simulink library "pne_pne3d_generic_std"  (R2016a)
(part 2 of 7)

      mask prompts: s1 "Solver Type: settings_iMode [-]"; s2 "Solver Step Size: settings_dt [s]"; initCmd "Initialization command"; p1 "Maximum Air Spring Level [mm] export=true name=dxMax prio=1 dataSetName=susp_dummy dataClassType=susp dataClassName=$dataSetClassAirSpring$ unit='mm' description='Maximum Air Spring Level [mm]': airSpring_Axle1.dxMax [-]"; p2 "Minimum Air Spring Level [mm] export=true name=dxMin prio=1 dataSetName=susp_dummy dataClassType=susp dataClassName=$dataSetClassAirSpring$ unit='mm' description='Minimum Air Spring Level [mm]': airSpring_Axle1.dxMin [-]"; p3 "Reference Lifting Displacement for dVRef [mm] export=true name=dxRef prio=1 dataSetName=susp_dummy dataClassType=susp dataClassName=$dataSetClassAirSpring$ unit='mm' description='Reference Lifting Displacement for dVRef [mm': airSpring_Axle1.dxRef [-]"; p4 "Lifting Speed [mm/s] export=true name=vLift prio=1 dataSetName=susp_dummy dataClassType=susp dataClassName=$dataSetClassAirSpring$ unit='mm/s' description='Lifting Speed [mm/s] ': airSpring_Axle1.vLift [-]"; p5 "Lowering Speed [mm/s] export=true name=vLow prio=1 dataSetName=susp_dummy dataClassType=susp dataClassName=$dataSetClassAirSpring$ unit='mm/s' description='Lowering Speed [mm/s] ': airSpring_Axle1.vLow [-]"; p6 "Maximum Air Spring Level [mm] export=true name=dxMax prio=1 dataSetName=susp_dummy dataClassType=susp dataClassName=$dataSetClassAirSpring$ unit='mm' description='Maximum Air Spring Level [mm]': airSpring_Axle2.dxMax [-]"; p7 "Minimum Air Spring Level [mm] export=true name=dxMin prio=1 dataSetName=susp_dummy dataClassType=susp dataClassName=$dataSetClassAirSpring$ unit='mm' description='Minimum Air Spring Level [mm]': airSpring_Axle2.dxMin [-]"; p8 "Reference Lifting Displacement for dVRef [mm] export=true name=dxRef prio=1 dataSetName=susp_dummy dataClassType=susp dataClassName=$dataSetClassAirSpring$ unit='mm' description='Reference Lifting Displacement for dVRef [mm': airSpring_Axle2.dxRef [-]"; p9 "Lifting Speed [mm/s] export=true name=vLift prio=1 dataSetName=susp_dummy dataClassType=susp dataClassName=$dataSetClassAirSpring$ unit='mm/s' description='Lifting Speed [mm/s] ': airSpring_Axle2.vLift [-]"; p10 "Lowering Speed [mm/s] export=true name=vLow prio=1 dataSetName=susp_dummy dataClassType=susp dataClassName=$dataSetClassAirSpring$ unit='mm/s' description='Lowering Speed [mm/s] ': airSpring_Axle2.vLow [-]"; p11 "Maximum Air Spring Level [mm] export=true name=dxMax prio=1 dataSetName=susp_dummy dataClassType=susp dataClassName=$dataSetClassAirSpring$ unit='mm' description='Maximum Air Spring Level [mm]': airSpring_Axle3.dxMax [-]"; p12 "Minimum Air Spring Level [mm] export=true name=dxMin prio=1 dataSetName=susp_dummy dataClassType=susp dataClassName=$dataSetClassAirSpring$ unit='mm' description='Minimum Air Spring Level [mm]': airSpring_Axle3.dxMin [-]"; p13 "Reference Lifting Displacement for dVRef [mm] export=true name=dxRef prio=1 dataSetName=susp_dummy dataClassType=susp dataClassName=$dataSetClassAirSpring$ unit='mm' description='Reference Lifting Displacement for dVRef [mm': airSpring_Axle3.dxRef [-]"; p14 "Lifting Speed [mm/s] export=true name=vLift prio=1 dataSetName=susp_dummy dataClassType=susp dataClassName=$dataSetClassAirSpring$ unit='mm/s' description='Lifting Speed [mm/s] ': airSpring_Axle3.vLift [-]"; p15 "Lowering Speed [mm/s] export=true name=vLow prio=1 dataSetName=susp_dummy dataClassType=susp dataClassName=$dataSetClassAirSpring$ unit='mm/s' description='Lowering Speed [mm/s] ': airSpring_Axle3.vLow [-]"; p16 "Maximum Air Spring Level [mm] export=true name=dxMax prio=1 dataSetName=susp_dummy dataClassType=susp dataClassName=$dataSetClassAirSpring$ unit='mm' description='Maximum Air Spring Level [mm]': airSpring_Axle4.dxMax [-]"; p17 "Minimum Air Spring Level [mm] export=true name=dxMin prio=1 dataSetName=susp_dummy dataClassType=susp dataClassName=$dataSetClassAirSpring$ unit='mm' description='Minimum Air Spring Level [mm]': airSpring_Axle4.dxMin [-]"; p18 "Reference Lifting Displacement for dVRef [mm] export=true name=dxRef prio=1 dataSetName=susp_dummy dataClassType=susp dataClassName=$dataSetClassAirSpring$ unit='mm' description='Reference Lifting Displacement for dVRef [mm': airSpring_Axle4.dxRef [-]"; p19 "Lifting Speed [mm/s] export=true name=vLift prio=1 dataSetName=susp_dummy dataClassType=susp dataClassName=$dataSetClassAirSpring$ unit='mm/s' description='Lifting Speed [mm/s] ': airSpring_Axle4.vLift [-]"; p20 "Lowering Speed [mm/s] export=true name=vLow prio=1 dataSetName=susp_dummy dataClassType=susp dataClassName=$dataSetClassAirSpring$ unit='mm/s' description='Lowering Speed [mm/s] ': airSpring_Axle4.vLow [-]"; p21 "Brake Type (Disc - 0, Drum - 1)  export=true name=brakeType prio=1 dataSetName=brk_dummy dataClassType=brk dataClassName=$dataSetClassBrk$ unit='-' description='Brake Type (Disc - 0, Drum - 1)': BrakeA1_R.brakeType [-]"; p22 "brake type dependent surface area [m^2] (C_TEM_A_NORM) export=true name=bt_A_norm prio=1 dataSetName=brk_dummy dataClassType=brk dataClassName=$dataSetClassBrk$  unit='m^2' description='brake type dependent surface area [m^2] (C_TEM_A_NORM)': BrakeA1_R.bt_A_norm [m²]"; p23 "brake pad friction area [m^2] export=true name=bt_A_pad prio=1 dataSetName=brk_dummy dataClassType=brk dataClassName=$dataSetClassBrk$  unit='m^2' description='brake pad friction area [m^2]': BrakeA1_R.bt_A_pad [m²]"; p24 "brake type dependent scaling for the heat loss due to convection at the cooling brake surface [-] (C_TEM_FAC_CONV_COOL) export=true name=bt_alpha_conv_fac_cool prio=1 dataSetName=brk_dummy dataClassType=brk dataClassName=$dataSetClassBrk$  unit='-' description='bbrake type dependent scaling for the heat loss due to convection at the cooling brake surface [-] (C_TEM_FAC_CONV_COOL)': BrakeA1_R.bt_alpha_conv_fac_cool [-]"; p25 "brake type dependent scaling for the heat loss due to convection at the friction brake surface [-] (C_TEM_FAC_CONV_FRIC) export=true name=bt_alpha_conv_fac_fric prio=1 dataSetName=brk_dummy dataClassType=brk dataClassName=$dataSetClassBrk$  unit='-' description='brake type dependent scaling for the heat loss due to convection at the friction brake surface [-] (C_TEM_FAC_CONV_FRIC)': BrakeA1_R.bt_alpha_conv_fac_fric [-]"; p26 "brake type dependent correction of heat loss due to conduction into the brake base [-] (C_TEM_CONDUCT_BASE) export=true name=bt_base_conduction_corr prio=1 dataSetName=brk_dummy dataClassType=brk dataClassName=$dataSetClassBrk$  unit='-' description='brake type dependent correction of heat loss due to conduction into the brake base [-] (C_TEM_CONDUCT_BASE)': BrakeA1_R.bt_base_conduction_corr [-]"; p27 "brake type dependent spatial discretization length [m] (C_TEM_DELTA_R) export=true name=bt_delta_r prio=1 dataSetName=brk_dummy dataClassType=brk dataClassName=$dataSetClassBrk$  unit='m' description='brake type dependent spatial discretization length [m] (C_TEM_DELTA_R)': BrakeA1_R.bt_delta_r [m]"; p28 "brake type dependent density correction [-] (C_TEM_DENSITY_CORR) export=true name=bt_density_correction prio=1 dataSetName=brk_dummy dataClassType=brk dataClassName=$dataSetClassBrk$  unit='-' description='brake type dependent density correction [-] (C_TEM_DENSITY_CORR)': BrakeA1_R.bt_density_correction [-]"; p29 "brake type dependent emission number [-] (C_TEM_EPSILON_BrakeType/C_TEM_EPSILON) export=true name=bt_epsilon_corr prio=1 dataSetName=brk_dummy dataClassType=brk dataClassName=$dataSetClassBrk$  unit='-' description='brake type dependent emission number [-] (C_TEM_EPSILON_BrakeType/C_TEM_EPSILON)': BrakeA1_R.bt_epsilon_corr [-]"; p30 "brake type dependent correction for cylindrical coordinates [-] (C_TEM_CYLINDER_CORR) export=true name=bt_rad_offset prio=1 dataSetName=brk_dummy dataClassType=brk dataClassName=$dataSetClassBrk$  unit='-' description='brake type dependent correction for cylindrical coordinates [-] (C_TEM_CYLINDER_CORR)': BrakeA1_R.bt_rad_offset [-]"; p31 "brake type dependent area correction for radiation [-] (C_TEM_RAD_AREA_CORR) export=true name=bt_radiation_area_corr prio=1 dataSetName=brk_dummy dataClassType=brk dataClassName=$dataSetClassBrk$  unit='-' description='brake type dependent area correction for radiation [-] (C_TEM_RAD_AREA_CORR)': BrakeA1_R.bt_radiation_area_corr [-]"; p32 "Consider Grinding Torque (0-false, 1-true) export=true name=considerTg prio=1 dataSetName=brk_dummy dataClassType=brk dataClassName=$dataSetClassBrk$  unit='-' description='Consider Grinding Torque (0-false, 1-true)': BrakeA1_R.considerTg [-]"; p33 "Brake Factor export=true name=Cs prio=1 dataSetName=brk_dummy dataClassType=brk dataClassName=$dataSetClassBrk$  unit='-' description='Brake Factor': BrakeA1_R.Cs [-]"; p34 "Efficiency export=true name=eta prio=1 dataSetName=brk_dummy dataClassType=brk dataClassName=$dataSetClassBrk$  unit='-' description='Efficiency': BrakeA1_R.eta [-]"; p35 "Dimension Temperature Correction Factor-Vector Length (max. 25) export=true name=fac_T_Dim prio=1 dataSetName=brk_dummy dataClassType=brk dataClassName=$dataSetClassBrk$  unit='-' description='Dimension Temperature Correction Factor-Vector Length (max. 25)': BrakeA1_R.fac_T_Dim [-]"; p36 "Dimension Velocity Correction Factor-Vector Length (max. 10) export=true name=fac_v_Dim prio=1 dataSetName=brk_dummy dataClassType=brk dataClassName=$dataSetClassBrk$  unit='-' description='Dimension Velocity Correction Factor-Vector Length (max. 10)': BrakeA1_R.fac_v_Dim [-]"; p37 "Dimension Fdx-Vector Length (max. 10) export=true name=Fdx_Dim prio=1 dataSetName=brk_dummy dataClassType=brk dataClassName=$dataSetClassBrk$  unit='-' description='Dimension Fdx-Vector Length (max. 10)': BrakeA1_R.Fdx_Dim [-]"; p38 "Gathering Factor Wear export=true name=Gwear prio=1 dataSetName=brk_dummy dataClassType=brk dataClassName=$dataSetClassBrk$  unit='-' description='Gathering Factor Wear': BrakeA1_R.Gwear [-]"; p39 "Dimension of i-dx-Vector Length (Transmission Ratio FBrake/FPiston) (max. 15) export=true name=i_Dim prio=1 dataSetName=brk_dummy dataClassType=brk dataClassName=$dataSetClassBrk$  unit='-' description='Dimension of i-dx-Vector Length (Transmission Ratio FBrake/FPiston) (max. 15)': BrakeA1_R.i_Dim [-]"; p40 "Effective Brake Radius export=true name=reff prio=1 dataSetName=brk_dummy dataClassType=brk dataClassName=$dataSetClassBrk$  unit='m' description='Effective Brake Radius': BrakeA1_R.reff [m]"; p41 "Initial Sum Brake Pad Thickness sPad_sum0 export=true name=sPad_sum0 prio=1 dataSetName=brk_dummy dataClassType=brk dataClassName=$dataSetClassBrk$  unit='m' description='Initial Sum Brake Pad Thickness sPad_sum0 [m]': BrakeA1_R.sPad_sum0 [m]"; p42 "Temperature calculation mode: 0 - constant temperature, 1 - variable temperature export=true name=useVarTempCalc prio=1 dataSetName=brk_dummy dataClassType=brk dataClassName=$dataSetClassBrk$  unit='-' description='Temperature calculation mode: 0 - constant temperature, 1 - variable temperature': BrakeA1_R.useVarTempCalc [-]"; p43 "Dimension Temperature Correction Factor-Vector Length (max. 20) export=true name=wearRate_T_Dim prio=1 dataSetName=brk_dummy dataClassType=brk dataClassName=$dataSetClassBrk$  unit='-' description='Dimension Temperature Correction Factor-Vector Length (max. 20)': BrakeA1_R.wearRate_T_Dim [-]"; p44 "Brake Type (Disc - 0, Drum - 1)  export=true name=brakeType prio=1 dataSetName=brk_dummy dataClassType=brk dataClassName=$dataSetClassBrk$ unit='-' description='Brake Type (Disc - 0, Drum - 1)': BrakeA2_R.brakeType [-]"; p45 "brake type dependent surface area [m^2] (C_TEM_A_NORM) export=true name=bt_A_norm prio=1 dataSetName=brk_dummy dataClassType=brk dataClassName=$dataSetClassBrk$  unit='m^2' description='brake type dependent surface area [m^2] (C_TEM_A_NORM)': BrakeA2_R.bt_A_norm [m²]"; p46 "brake pad friction area [m^2] export=true name=bt_A_pad prio=1 dataSetName=brk_dummy dataClassType=brk dataClassName=$dataSetClassBrk$  unit='m^2' description='brake pad friction area [m^2]': BrakeA2_R.bt_A_pad [m²]"; p47 "brake type dependent scaling for the heat loss due to convection at the cooling brake surface [-] (C_TEM_FAC_CONV_COOL) export=true name=bt_alpha_conv_fac_cool prio=1 dataSetName=brk_dummy dataClassType=brk dataClassName=$dataSetClassBrk$  unit='-' description='bbrake type dependent scaling for the heat loss due to convection at the cooling brake surface [-] (C_TEM_FAC_CONV_COOL)': BrakeA2_R.bt_alpha_conv_fac_cool [-]"; p48 "brake type dependent scaling for the heat loss due to convection at the friction brake surface [-] (C_TEM_FAC_CONV_FRIC) export=true name=bt_alpha_conv_fac_fric prio=1 dataSetName=brk_dummy dataClassType=brk dataClassName=$dataSetClassBrk$  unit='-' description='brake type dependent scaling for the heat loss due to convection at the friction brake surface [-] (C_TEM_FAC_CONV_FRIC)': BrakeA2_R.bt_alpha_conv_fac_fric [-]"; p49 "brake type dependent correction of heat loss due to conduction into the brake base [-] (C_TEM_CONDUCT_BASE) export=true name=bt_base_conduction_corr prio=1 dataSetName=brk_dummy dataClassType=brk dataClassName=$dataSetClassBrk$  unit='-' description='brake type dependent correction of heat loss due to conduction into the brake base [-] (C_TEM_CONDUCT_BASE)': BrakeA2_R.bt_base_conduction_corr [-]"; p50 "brake type dependent spatial discretization length [m] (C_TEM_DELTA_R) export=true name=bt_delta_r prio=1 dataSetName=brk_dummy dataClassType=brk dataClassName=$dataSetClassBrk$  unit='m' description='brake type dependent spatial discretization length [m] (C_TEM_DELTA_R)': BrakeA2_R.bt_delta_r [m]"; p51 "brake type dependent density correction [-] (C_TEM_DENSITY_CORR) export=true name=bt_density_correction prio=1 dataSetName=brk_dummy dataClassType=brk dataClassName=$dataSetClassBrk$  unit='-' description='brake type dependent density correction [-] (C_TEM_DENSITY_CORR)': BrakeA2_R.bt_density_correction [-]"; p52 "brake type dependent emission number [-] (C_TEM_EPSILON_BrakeType/C_TEM_EPSILON) export=true name=bt_epsilon_corr prio=1 dataSetName=brk_dummy dataClassType=brk dataClassName=$dataSetClassBrk$  unit='-' description='brake type dependent emission number [-] (C_TEM_EPSILON_BrakeType/C_TEM_EPSILON)': BrakeA2_R.bt_epsilon_corr [-]"; p53 "brake type dependent correction for cylindrical coordinates [-] (C_TEM_CYLINDER_CORR) export=true name=bt_rad_offset prio=1 dataSetName=brk_dummy dataClassType=brk dataClassName=$dataSetClassBrk$  unit='-' description='brake type dependent correction for cylindrical coordinates [-] (C_TEM_CYLINDER_CORR)': BrakeA2_R.bt_rad_offset [-]"; p54 "brake type dependent area correction for radiation [-] (C_TEM_RAD_AREA_CORR) export=true name=bt_radiation_area_corr prio=1 dataSetName=brk_dummy dataClassType=brk dataClassName=$dataSetClassBrk$  unit='-' description='brake type dependent area correction for radiation [-] (C_TEM_RAD_AREA_CORR)': BrakeA2_R.bt_radiation_area_corr [-]"; p55 "Consider Grinding Torque (0-false, 1-true) export=true name=considerTg prio=1 dataSetName=brk_dummy dataClassType=brk dataClassName=$dataSetClassBrk$  unit='-' description='Consider Grinding Torque (0-false, 1-true)': BrakeA2_R.considerTg [-]"; p56 "Brake Factor export=true name=Cs prio=1 dataSetName=brk_dummy dataClassType=brk dataClassName=$dataSetClassBrk$  unit='-' description='Brake Factor': BrakeA2_R.Cs [-]"; p57 "Efficiency export=true name=eta prio=1 dataSetName=brk_dummy dataClassType=brk dataClassName=$dataSetClassBrk$  unit='-' description='Efficiency': BrakeA2_R.eta [-]"; p58 "Dimension Temperature Correction Factor-Vector Length (max. 25) export=true name=fac_T_Dim prio=1 dataSetName=brk_dummy dataClassType=brk dataClassName=$dataSetClassBrk$  unit='-' description='Dimension Temperature Correction Factor-Vector Length (max. 25)': BrakeA2_R.fac_T_Dim [-]"; p59 "Dimension Velocity Correction Factor-Vector Length (max. 10) export=true name=fac_v_Dim prio=1 dataSetName=brk_dummy dataClassType=brk dataClassName=$dataSetClassBrk$  unit='-' description='Dimension Velocity Correction Factor-Vector Length (max. 10)': BrakeA2_R.fac_v_Dim [-]"; p60 "Dimension Fdx-Vector Length (max. 10) export=true name=Fdx_Dim prio=1 dataSetName=brk_dummy dataClassType=brk dataClassName=$dataSetClassBrk$  unit='-' description='Dimension Fdx-Vector Length (max. 10)': BrakeA2_R.Fdx_Dim [-]"; p61 "Gathering Factor Wear export=true name=Gwear prio=1 dataSetName=brk_dummy dataClassType=brk dataClassName=$dataSetClassBrk$  unit='-' description='Gathering Factor Wear': BrakeA2_R.Gwear [-]"; p62 "Dimension of i-dx-Vector Length (Transmission Ratio FBrake/FPiston) (max. 15) export=true name=i_Dim prio=1 dataSetName=brk_dummy dataClassType=brk dataClassName=$dataSetClassBrk$  unit='-' description='Dimension of i-dx-Vector Length (Transmission Ratio FBrake/FPiston) (max. 15)': BrakeA2_R.i_Dim [-]"; p63 "Effective Brake Radius export=true name=reff prio=1 dataSetName=brk_dummy dataClassType=brk dataClassName=$dataSetClassBrk$  unit='m' description='Effective Brake Radius': BrakeA2_R.reff [m]"; p64 "Initial Sum Brake Pad Thickness sPad_sum0 export=true name=sPad_sum0 prio=1 dataSetName=brk_dummy dataClassType=brk dataClassName=$dataSetClassBrk$  unit='m' description='Initial Sum Brake Pad Thickness sPad_sum0 [m]': BrakeA2_R.sPad_sum0 [m]"; p65 "Temperature calculation mode: 0 - constant temperature, 1 - variable temperature export=true name=useVarTempCalc prio=1 dataSetName=brk_dummy dataClassType=brk dataClassName=$dataSetClassBrk$  unit='-' description='Temperature calculation mode: 0 - constant temperature, 1 - variable temperature': BrakeA2_R.useVarTempCalc [-]"; p66 "Dimension Temperature Correction Factor-Vector Length (max. 20) export=true name=wearRate_T_Dim prio=1 dataSetName=brk_dummy dataClassType=brk dataClassName=$dataSetClassBrk$  unit='-' description='Dimension Temperature Correction Factor-Vector Length (max. 20)': BrakeA2_R.wearRate_T_Dim [-]"; p67 "Brake Type (Disc - 0, Drum - 1)  export=true name=brakeType prio=1 dataSetName=brk_dummy dataClassType=brk dataClassName=$dataSetClassBrk$ unit='-' description='Brake Type (Disc - 0, Drum - 1)': BrakeA3_R.brakeType [-]"; p68 "brake type dependent surface area [m^2] (C_TEM_A_NORM) export=true name=bt_A_norm prio=1 dataSetName=brk_dummy dataClassType=brk dataClassName=$dataSetClassBrk$  unit='m^2' description='brake type dependent surface area [m^2] (C_TEM_A_NORM)': BrakeA3_R.bt_A_norm [m²]"; p69 "brake pad friction area [m^2] export=true name=bt_A_pad prio=1 dataSetName=brk_dummy dataClassType=brk dataClassName=$dataSetClassBrk$  unit='m^2' description='brake pad friction area [m^2]': BrakeA3_R.bt_A_pad [m²]"; p70 "brake type dependent scaling for the heat loss due to convection at the cooling brake surface [-] (C_TEM_FAC_CONV_COOL) export=true name=bt_alpha_conv_fac_cool prio=1 dataSetName=brk_dummy dataClassType=brk dataClassName=$dataSetClassBrk$  unit='-' description='bbrake type dependent scaling for the heat loss due to convection at the cooling brake surface [-] (C_TEM_FAC_CONV_COOL)': BrakeA3_R.bt_alpha_conv_fac_cool [-]"; p71 "brake type dependent scaling for the heat loss due to convection at the friction brake surface [-] (C_TEM_FAC_CONV_FRIC) export=true name=bt_alpha_conv_fac_fric prio=1 dataSetName=brk_dummy dataClassType=brk dataClassName=$dataSetClassBrk$  unit='-' description='brake type dependent scaling for the heat loss due to convection at the friction brake surface [-] (C_TEM_FAC_CONV_FRIC)': BrakeA3_R.bt_alpha_conv_fac_fric [-]"; p72 "brake type dependent correction of heat loss due to conduction into the brake base [-] (C_TEM_CONDUCT_BASE) export=true name=bt_base_conduction_corr prio=1 dataSetName=brk_dummy dataClassType=brk dataClassName=$dataSetClassBrk$  unit='-' description='brake type dependent correction of heat loss due to conduction into the brake base [-] (C_TEM_CONDUCT_BASE)': BrakeA3_R.bt_base_conduction_corr [-]"; p73 "brake type dependent spatial discretization length [m] (C_TEM_DELTA_R) export=true name=bt_delta_r prio=1 dataSetName=brk_dummy dataClassType=brk dataClassName=$dataSetClassBrk$  unit='m' description='brake type dependent spatial discretization length [m] (C_TEM_DELTA_R)': BrakeA3_R.bt_delta_r [m]"; p74 "brake type dependent density correction [-] (C_TEM_DENSITY_CORR) export=true name=bt_density_correction prio=1 dataSetName=brk_dummy dataClassType=brk dataClassName=$dataSetClassBrk$  unit='-' description='brake type dependent density correction [-] (C_TEM_DENSITY_CORR)': BrakeA3_R.bt_density_correction [-]"; p75 "brake type dependent emission number [-] (C_TEM_EPSILON_BrakeType/C_TEM_EPSILON) export=true name=bt_epsilon_corr prio=1 dataSetName=brk_dummy dataClassType=brk dataClassName=$dataSetClassBrk$  unit='-' description='brake type dependent emission number [-] (C_TEM_EPSILON_BrakeType/C_TEM_EPSILON)': BrakeA3_R.bt_epsilon_corr [-]"; p76 "brake type dependent correction for cylindrical coordinates [-] (C_TEM_CYLINDER_CORR) export=true name=bt_rad_offset prio=1 dataSetName=brk_dummy dataClassType=brk dataClassName=$dataSetClassBrk$  unit='-' description='brake type dependent correction for cylindrical coordinates [-] (C_TEM_CYLINDER_CORR)': BrakeA3_R.bt_rad_offset [-]"; p77 "brake type dependent area correction for radiation [-] (C_TEM_RAD_AREA_CORR) export=true name=bt_radiation_area_corr prio=1 dataSetName=brk_dummy dataClassType=brk dataClassName=$dataSetClassBrk$  unit='-' description='brake type dependent area correction for radiation [-] (C_TEM_RAD_AREA_CORR)': BrakeA3_R.bt_radiation_area_corr [-]"; p78 "Consider Grinding Torque (0-false, 1-true) export=true name=considerTg prio=1 dataSetName=brk_dummy dataClassType=brk dataClassName=$dataSetClassBrk$  unit='-' description='Consider Grinding Torque (0-false, 1-true)': BrakeA3_R.considerTg [-]"; p79 "Brake Factor export=true name=Cs prio=1 dataSetName=brk_dummy dataClassType=brk dataClassName=$dataSetClassBrk$  unit='-' description='Brake Factor': BrakeA3_R.Cs [-]"; p80 "Efficiency export=true name=eta prio=1 dataSetName=brk_dummy dataClassType=brk dataClassName=$dataSetClassBrk$  unit='-' description='Efficiency': BrakeA3_R.eta [-]"; p81 "Dimension Temperature Correction Factor-Vector Length (max. 25) export=true name=fac_T_Dim prio=1 dataSetName=brk_dummy dataClassType=brk dataClassName=$dataSetClassBrk$  unit='-' description='Dimension Temperature Correction Factor-Vector Length (max. 25)': BrakeA3_R.fac_T_Dim [-]"; p82 "Dimension Velocity Correction Factor-Vector Length (max. 10) export=true name=fac_v_Dim prio=1 dataSetName=brk_dummy dataClassType=brk dataClassName=$dataSetClassBrk$  unit='-' description='Dimension Velocity Correction Factor-Vector Length (max. 10)': BrakeA3_R.fac_v_Dim [-]"; p83 "Dimension Fdx-Vector Length (max. 10) export=true name=Fdx_Dim prio=1 dataSetName=brk_dummy dataClassType=brk dataClassName=$dataSetClassBrk$  unit='-' description='Dimension Fdx-Vector Length (max. 10)': BrakeA3_R.Fdx_Dim [-]"; p84 "Gathering Factor Wear export=true name=Gwear prio=1 dataSetName=brk_dummy dataClassType=brk dataClassName=$dataSetClassBrk$  unit='-' description='Gathering Factor Wear': BrakeA3_R.Gwear [-]"; p85 "Dimension of i-dx-Vector Length (Transmission Ratio FBrake/FPiston) (max. 15) export=true name=i_Dim prio=1 dataSetName=brk_dummy dataClassType=brk dataClassName=$dataSetClassBrk$  unit='-' description='Dimension of i-dx-Vector Length (Transmission Ratio FBrake/FPiston) (max. 15)': BrakeA3_R.i_Dim [-]"; p86 "Effective Brake Radius export=true name=reff prio=1 dataSetName=brk_dummy dataClassType=brk dataClassName=$dataSetClassBrk$  unit='m' description='Effective Brake Radius': BrakeA3_R.reff [m]"; p87 "Initial Sum Brake Pad Thickness sPad_sum0 export=true name=sPad_sum0 prio=1 dataSetName=brk_dummy dataClassType=brk dataClassName=$dataSetClassBrk$  unit='m' description='Initial Sum Brake Pad Thickness sPad_sum0 [m]': BrakeA3_R.sPad_sum0 [m]"; p88 "Temperature calculation mode: 0 - constant temperature, 1 - variable temperature export=true name=useVarTempCalc prio=1 dataSetName=brk_dummy dataClassType=brk dataClassName=$dataSetClassBrk$  unit='-' description='Temperature calculation mode: 0 - constant temperature, 1 - variable temperature': BrakeA3_R.useVarTempCalc [-]"; p89 "Dimension Temperature Correction Factor-Vector Length (max. 20) export=true name=wearRate_T_Dim prio=1 dataSetName=brk_dummy dataClassType=brk dataClassName=$dataSetClassBrk$  unit='-' description='Dimension Temperature Correction Factor-Vector Length (max. 20)': BrakeA3_R.wearRate_T_Dim [-]"; p90 "Brake Type (Disc - 0, Drum - 1)  export=true name=brakeType prio=1 dataSetName=brk_dummy dataClassType=brk dataClassName=$dataSetClassBrk$ unit='-' description='Brake Type (Disc - 0, Drum - 1)': BrakeA4_R.brakeType [-]"; p91 "brake type dependent surface area [m^2] (C_TEM_A_NORM) export=true name=bt_A_norm prio=1 dataSetName=brk_dummy dataClassType=brk dataClassName=$dataSetClassBrk$  unit='m^2' description='brake type dependent surface area [m^2] (C_TEM_A_NORM)': BrakeA4_R.bt_A_norm [m²]"; p92 "brake pad friction area [m^2] export=true name=bt_A_pad prio=1 dataSetName=brk_dummy dataClassType=brk dataClassName=$dataSetClassBrk$  unit='m^2' description='brake pad friction area [m^2]': BrakeA4_R.bt_A_pad [m²]"; p93 "brake type dependent scaling for the heat loss due to convection at the cooling brake surface [-] (C_TEM_FAC_CONV_COOL) export=true name=bt_alpha_conv_fac_cool prio=1 dataSetName=brk_dummy dataClassType=brk dataClassName=$dataSetClassBrk$  unit='-' description='bbrake type dependent scaling for the heat loss due to convection at the cooling brake surface [-] (C_TEM_FAC_CONV_COOL)': BrakeA4_R.bt_alpha_conv_fac_cool [-]"; p94 "brake type dependent scaling for the heat loss due to convection at the friction brake surface [-] (C_TEM_FAC_CONV_FRIC) export=true name=bt_alpha_conv_fac_fric prio=1 dataSetName=brk_dummy dataClassType=brk dataClassName=$dataSetClassBrk$  unit='-' description='brake type dependent scaling for the heat loss due to convection at the friction brake surface [-] (C_TEM_FAC_CONV_FRIC)': BrakeA4_R.bt_alpha_conv_fac_fric [-]"; p95 "brake type dependent correction of heat loss due to conduction into the brake base [-] (C_TEM_CONDUCT_BASE) export=true name=bt_base_conduction_corr prio=1 dataSetName=brk_dummy dataClassType=brk dataClassName=$dataSetClassBrk$  unit='-' description='brake type dependent correction of heat loss due to conduction into the brake base [-] (C_TEM_CONDUCT_BASE)': BrakeA4_R.bt_base_conduction_corr [-]"; p96 "brake type dependent spatial discretization length [m] (C_TEM_DELTA_R) export=true name=bt_delta_r prio=1 dataSetName=brk_dummy dataClassType=brk dataClassName=$dataSetClassBrk$  unit='m' description='brake type dependent spatial discretization length [m] (C_TEM_DELTA_R)': BrakeA4_R.bt_delta_r [m]"; p97 "brake type dependent density correction [-] (C_TEM_DENSITY_CORR) export=true name=bt_density_correction prio=1 dataSetName=brk_dummy dataClassType=brk dataClassName=$dataSetClassBrk$  unit='-' description='brake type dependent density correction [-] (C_TEM_DENSITY_CORR)': BrakeA4_R.bt_density_correction [-]"; p98 "brake type dependent emission number [-] (C_TEM_EPSILON_BrakeType/C_TEM_EPSILON) export=true name=bt_epsilon_corr prio=1 dataSetName=brk_dummy dataClassType=brk dataClassName=$dataSetClassBrk$  unit='-' description='brake type dependent emission number [-] (C_TEM_EPSILON_BrakeType/C_TEM_EPSILON)': BrakeA4_R.bt_epsilon_corr [-]"; p99 "brake type dependent correction for cylindrical coordinates [-] (C_TEM_CYLINDER_CORR) export=true name=bt_rad_offset prio=1 dataSetName=brk_dummy dataClassType=brk dataClassName=$dataSetClassBrk$  unit='-' description='brake type dependent correction for cylindrical coordinates [-] (C_TEM_CYLINDER_CORR)': BrakeA4_R.bt_rad_offset [-]"; p100 "brake type dependent area correction for radiation [-] (C_TEM_RAD_AREA_CORR) export=true name=bt_radiation_area_corr prio=1 dataSetName=brk_dummy dataClassType=brk dataClassName=$dataSetClassBrk$  unit='-' description='brake type dependent area correction for radiation [-] (C_TEM_RAD_AREA_CORR)': BrakeA4_R.bt_radiation_area_corr [-]"; p101 "Consider Grinding Torque (0-false, 1-true) export=true name=considerTg prio=1 dataSetName=brk_dummy dataClassType=brk dataClassName=$dataSetClassBrk$  unit='-' description='Consider Grinding Torque (0-false, 1-true)': BrakeA4_R.considerTg [-]"; p102 "Brake Factor export=true name=Cs prio=1 dataSetName=brk_dummy dataClassType=brk dataClassName=$dataSetClassBrk$  unit='-' description='Brake Factor': BrakeA4_R.Cs [-]"; p103 "Efficiency export=true name=eta prio=1 dataSetName=brk_dummy dataClassType=brk dataClassName=$dataSetClassBrk$  unit='-' description='Efficiency': BrakeA4_R.eta [-]"; p104 "Dimension Temperature Correction Factor-Vector Length (max. 25) export=true name=fac_T_Dim prio=1 dataSetName=brk_dummy dataClassType=brk dataClassName=$dataSetClassBrk$  unit='-' description='Dimension Temperature Correction Factor-Vector Length (max. 25)': BrakeA4_R.fac_T_Dim [-]"; p105 "Dimension Velocity Correction Factor-Vector Length (max. 10) export=true name=fac_v_Dim prio=1 dataSetName=brk_dummy dataClassType=brk dataClassName=$dataSetClassBrk$  unit='-' description='Dimension Velocity Correction Factor-Vector Length (max. 10)': BrakeA4_R.fac_v_Dim [-]"; p106 "Dimension Fdx-Vector Length (max. 10) export=true name=Fdx_Dim prio=1 dataSetName=brk_dummy dataClassType=brk dataClassName=$dataSetClassBrk$  unit='-' description='Dimension Fdx-Vector Length (max. 10)': BrakeA4_R.Fdx_Dim [-]"; p107 "Gathering Factor Wear export=true name=Gwear prio=1 dataSetName=brk_dummy dataClassType=brk dataClassName=$dataSetClassBrk$  unit='-' description='Gathering Factor Wear': BrakeA4_R.Gwear [-]"; p108 "Dimension of i-dx-Vector Length (Transmission Ratio FBrake/FPiston) (max. 15) export=true name=i_Dim prio=1 dataSetName=brk_dummy dataClassType=brk dataClassName=$dataSetClassBrk$  unit='-' description='Dimension of i-dx-Vector Length (Transmission Ratio FBrake/FPiston) (max. 15)': BrakeA4_R.i_Dim [-]"; p109 "Effective Brake Radius export=true name=reff prio=1 dataSetName=brk_dummy dataClassType=brk dataClassName=$dataSetClassBrk$  unit='m' description='Effective Brake Radius': BrakeA4_R.reff [m]"; p110 "Initial Sum Brake Pad Thickness sPad_sum0 export=true name=sPad_sum0 prio=1 dataSetName=brk_dummy dataClassType=brk dataClassName=$dataSetClassBrk$  unit='m' description='Initial Sum Brake Pad Thickness sPad_sum0 [m]': BrakeA4_R.sPad_sum0 [m]"; p111 "Temperature calculation mode: 0 - constant temperature, 1 - variable temperature export=true name=useVarTempCalc prio=1 dataSetName=brk_dummy dataClassType=brk dataClassName=$dataSetClassBrk$  unit='-' description='Temperature calculation mode: 0 - constant temperature, 1 - variable temperature': BrakeA4_R.useVarTempCalc [-]"; p112 "Dimension Temperature Correction Factor-Vector Length (max. 20) export=true name=wearRate_T_Dim prio=1 dataSetName=brk_dummy dataClassType=brk dataClassName=$dataSetClassBrk$  unit='-' description='Dimension Temperature Correction Factor-Vector Length (max. 20)': BrakeA4_R.wearRate_T_Dim [-]"; p113 "Dimension of Parking Brake Spring Curve (max 10) export=true name=dxFSpring_Dim prio=1 dataSetName=cyl_dummy dataClassType=cyl dataClassName=$dataSetClassCyl$  unit='-' description='Dimension of Parking Brake Spring Curve (max 10)': brakeCylinderA1_R.dxFSpring_Dim [-]"; p114 "Dimension of Parking Brake Chamber Volume Curve (max 10) export=true name=dxVolPB_Dim prio=1 dataSetName=cyl_dummy dataClassType=cyl dataClassName=$dataSetClassCyl$  unit='-' description='Dimension of Parking Brake Chamber Volume Curve (max 10)': brakeCylinderA1_R.dxVolPB_Dim [-]"; p115 "Dimension of Service Brake Chamber Volume Curve (max 10) export=true name=dxVolSB_Dim prio=1 dataSetName=cyl_dummy dataClassType=cyl dataClassName=$dataSetClassCyl$  unit='-' description='Dimension of Service Brake Chamber Volume Curve (max 10)': brakeCylinderA1_R.dxVolSB_Dim [-]"; p116 "Nominal Force Membrane Cylinder at pNom export=true name=FNom prio=1 dataSetName=cyl_dummy dataClassType=cyl dataClassName=$dataSetClassCyl$ unit='N' description='Nominal Force Membrane Cylinder at pNom': brakeCylinderA1_R.FNom [N]"; p117 "Maximum Cylinder Stroke export=true name=maxStroke prio=1 dataSetName=cyl_dummy dataClassType=cyl dataClassName=$dataSetClassCyl$ unit='m' description='Maximum Cylinder Stroke': brakeCylinderA1_R.maxStroke [m]"; p118 "Application Pressure Membrane Chamber (relative to pAtm) export=true name=pApp prio=1 dataSetName=cyl_dummy dataClassType=cyl dataClassName=$dataSetClassCyl$  unit='Pa' description='Application Pressure Membrane Chamber (relative to pAtm)': brakeCylinderA1_R.pApp [Pa]"; p119 "Nominal Pressure (relative to pAtm) export=true name=pNom prio=1 dataSetName=cyl_dummy dataClassType=cyl dataClassName=$dataSetClassCyl$ unit='Pa' description='Nominal Pressure (relative to pAtm)': brakeCylinderA1_R.pNom [Pa]"; p120 "Spring Brake Release Pressure (relative to pAtm) export=true name=pR_PB prio=1 dataSetName=cyl_dummy dataClassType=cyl dataClassName=$dataSetClassCyl$ unit='Pa' description='Spring Brake Release Pressure (relative to pAtm)': brakeCylinderA1_R.pR_PB [Pa]"; p121 "Spring Brake Release Stroke at pR_PB export=true name=xR_PB prio=1 dataSetName=cyl_dummy dataClassType=cyl dataClassName=$dataSetClassCyl$ unit='m' description='Spring Brake Release Stroke at pR_PB': brakeCylinderA1_R.xR_PB [m]"; p122 "Dimension of Parking Brake Spring Curve (max 10) export=true name=dxFSpring_Dim prio=1 dataSetName=cyl_dummy dataClassType=cyl dataClassName=$dataSetClassCyl$  unit='-' description='Dimension of Parking Brake Spring Curve (max 10)': brakeCylinderA2_R.dxFSpring_Dim [-]"; p123 "Dimension of Parking Brake Chamber Volume Curve (max 10) export=true name=dxVolPB_Dim prio=1 dataSetName=cyl_dummy dataClassType=cyl dataClassName=$dataSetClassCyl$  unit='-' description='Dimension of Parking Brake Chamber Volume Curve (max 10)': brakeCylinderA2_R.dxVolPB_Dim [-]"; p124 "Dimension of Service Brake Chamber Volume Curve (max 10) export=true name=dxVolSB_Dim prio=1 dataSetName=cyl_dummy dataClassType=cyl dataClassName=$dataSetClassCyl$  unit='-' description='Dimension of Service Brake Chamber Volume Curve (max 10)': brakeCylinderA2_R.dxVolSB_Dim [-]"; p125 "Nominal Force Membrane Cylinder at pNom export=true name=FNom prio=1 dataSetName=cyl_dummy dataClassType=cyl dataClassName=$dataSetClassCyl$ unit='N' description='Nominal Force Membrane Cylinder at pNom': brakeCylinderA2_R.FNom [N]"; p126 "Maximum Cylinder Stroke export=true name=maxStroke prio=1 dataSetName=cyl_dummy dataClassType=cyl dataClassName=$dataSetClassCyl$ unit='m' description='Maximum Cylinder Stroke': brakeCylinderA2_R.maxStroke [m]"; p127 "Application Pressure Membrane Chamber (relative to pAtm) export=true name=pApp prio=1 dataSetName=cyl_dummy dataClassType=cyl dataClassName=$dataSetClassCyl$  unit='Pa' description='Application Pressure Membrane Chamber (relative to pAtm)': brakeCylinderA2_R.pApp [Pa]"; p128 "Nominal Pressure (relative to pAtm) export=true name=pNom prio=1 dataSetName=cyl_dummy dataClassType=cyl dataClassName=$dataSetClassCyl$ unit='Pa' description='Nominal Pressure (relative to pAtm)': brakeCylinderA2_R.pNom [Pa]"; p129 "Spring Brake Release Pressure (relative to pAtm) export=true name=pR_PB prio=1 dataSetName=cyl_dummy dataClassType=cyl dataClassName=$dataSetClassCyl$ unit='Pa' description='Spring Brake Release Pressure (relative to pAtm)': brakeCylinderA2_R.pR_PB [Pa]"; p130 "Spring Brake Release Stroke at pR_PB export=true name=xR_PB prio=1 dataSetName=cyl_dummy dataClassType=cyl dataClassName=$dataSetClassCyl$ unit='m' description='Spring Brake Release Stroke at pR_PB': brakeCylinderA2_R.xR_PB [m]"; p131 "Dimension of Parking Brake Spring Curve (max 10) export=true name=dxFSpring_Dim prio=1 dataSetName=cyl_dummy dataClassType=cyl dataClassName=$dataSetClassCyl$  unit='-' description='Dimension of Parking Brake Spring Curve (max 10)': brakeCylinderA3_R.dxFSpring_Dim [-]"; p132 "Dimension of Parking Brake Chamber Volume Curve (max 10) export=true name=dxVolPB_Dim prio=1 dataSetName=cyl_dummy dataClassType=cyl dataClassName=$dataSetClassCyl$  unit='-' description='Dimension of Parking Brake Chamber Volume Curve (max 10)': brakeCylinderA3_R.dxVolPB_Dim [-]"; p133 "Dimension of Service Brake Chamber Volume Curve (max 10) export=true name=dxVolSB_Dim prio=1 dataSetName=cyl_dummy dataClassType=cyl dataClassName=$dataSetClassCyl$  unit='-' description='Dimension of Service Brake Chamber Volume Curve (max 10)': brakeCylinderA3_R.dxVolSB_Dim [-]"; p134 "Nominal Force Membrane Cylinder at pNom export=true name=FNom prio=1 dataSetName=cyl_dummy dataClassType=cyl dataClassName=$dataSetClassCyl$ unit='N' description='Nominal Force Membrane Cylinder at pNom': brakeCylinderA3_R.FNom [N]"; p135 "Maximum Cylinder Stroke export=true name=maxStroke prio=1 dataSetName=cyl_dummy dataClassType=cyl dataClassName=$dataSetClassCyl$ unit='m' description='Maximum Cylinder Stroke': brakeCylinderA3_R.maxStroke [m]"; p136 "Application Pressure Membrane Chamber (relative to pAtm) export=true name=pApp prio=1 dataSetName=cyl_dummy dataClassType=cyl dataClassName=$dataSetClassCyl$  unit='Pa' description='Application Pressure Membrane Chamber (relative to pAtm)': brakeCylinderA3_R.pApp [Pa]"; p137 "Nominal Pressure (relative to pAtm) export=true name=pNom prio=1 dataSetName=cyl_dummy dataClassType=cyl dataClassName=$dataSetClassCyl$ unit='Pa' description='Nominal Pressure (relative to pAtm)': brakeCylinderA3_R.pNom [Pa]"; p138 "Spring Brake Release Pressure (relative to pAtm) export=true name=pR_PB prio=1 dataSetName=cyl_dummy dataClassType=cyl dataClassName=$dataSetClassCyl$ unit='Pa' description='Spring Brake Release Pressure (relative to pAtm)': brakeCylinderA3_R.pR_PB [Pa]"; p139 "Spring Brake Release Stroke at pR_PB export=true name=xR_PB prio=1 dataSetName=cyl_dummy dataClassType=cyl dataClassName=$dataSetClassCyl$ unit='m' description='Spring Brake Release Stroke at pR_PB': brakeCylinderA3_R.xR_PB [m]"; p140 "Dimension of Parking Brake Spring Curve (max 10) export=true name=dxFSpring_Dim prio=1 dataSetName=cyl_dummy dataClassType=cyl dataClassName=$dataSetClassCyl$  unit='-' description='Dimension of Parking Brake Spring Curve (max 10)': brakeCylinderA4_R.dxFSpring_Dim [-]"; p141 "Dimension of Parking Brake Chamber Volume Curve (max 10) export=true name=dxVolPB_Dim prio=1 dataSetName=cyl_dummy dataClassType=cyl dataClassName=$dataSetClassCyl$  unit='-' description='Dimension of Parking Brake Chamber Volume Curve (max 10)': brakeCylinderA4_R.dxVolPB_Dim [-]"; p142 "Dimension of Service Brake Chamber Volume Curve (max 10) export=true name=dxVolSB_Dim prio=1 dataSetName=cyl_dummy dataClassType=cyl dataClassName=$dataSetClassCyl$  unit='-' description='Dimension of Service Brake Chamber Volume Curve (max 10)': brakeCylinderA4_R.dxVolSB_Dim [-]"; p143 "Nominal Force Membrane Cylinder at pNom export=true name=FNom prio=1 dataSetName=cyl_dummy dataClassType=cyl dataClassName=$dataSetClassCyl$ unit='N' description='Nominal Force Membrane Cylinder at pNom': brakeCylinderA4_R.FNom [N]"; p144 "Maximum Cylinder Stroke export=true name=maxStroke prio=1 dataSetName=cyl_dummy dataClassType=cyl dataClassName=$dataSetClassCyl$ unit='m' description='Maximum Cylinder Stroke': brakeCylinderA4_R.maxStroke [m]"; p145 "Application Pressure Membrane Chamber (relative to pAtm) export=true name=pApp prio=1 dataSetName=cyl_dummy dataClassType=cyl dataClassName=$dataSetClassCyl$  unit='Pa' description='Application Pressure Membrane Chamber (relative to pAtm)': brakeCylinderA4_R.pApp [Pa]"; p146 "Nominal Pressure (relative to pAtm) export=true name=pNom prio=1 dataSetName=cyl_dummy dataClassType=cyl dataClassName=$dataSetClassCyl$ unit='Pa' description='Nominal Pressure (relative to pAtm)': brakeCylinderA4_R.pNom [Pa]"; p147 "Spring Brake Release Pressure (relative to pAtm) export=true name=pR_PB prio=1 dataSetName=cyl_dummy dataClassType=cyl dataClassName=$dataSetClassCyl$ unit='Pa' description='Spring Brake Release Pressure (relative to pAtm)': brakeCylinderA4_R.pR_PB [Pa]"; p148 "Spring Brake Release Stroke at pR_PB export=true name=xR_PB prio=1 dataSetName=cyl_dummy dataClassType=cyl dataClassName=$dataSetClassCyl$ unit='m' description='Spring Brake Release Stroke at pR_PB': brakeCylinderA4_R.xR_PB [m]"; p149 "Dimension of Parking Brake Spring Curve (max 10) export=true name=dxFSpring_Dim prio=1 dataSetName=cyl_dummy dataClassType=cyl dataClassName=$dataSetClassCyl$  unit='-' description='Dimension of Parking Brake Spring Curve (max 10)': brakeCylinderTrailerA1_R.dxFSpring_Dim [-]"; p150 "Dimension of Parking Brake Chamber Volume Curve (max 10) export=true name=dxVolPB_Dim prio=1 dataSetName=cyl_dummy dataClassType=cyl dataClassName=$dataSetClassCyl$  unit='-' description='Dimension of Parking Brake Chamber Volume Curve (max 10)': brakeCylinderTrailerA1_R.dxVolPB_Dim [-]"; p151 "Dimension of Service Brake Chamber Volume Curve (max 10) export=true name=dxVolSB_Dim prio=1 dataSetName=cyl_dummy dataClassType=cyl dataClassName=$dataSetClassCyl$  unit='-' description='Dimension of Service Brake Chamber Volume Curve (max 10)': brakeCylinderTrailerA1_R.dxVolSB_Dim [-]"; p152 "Nominal Force Membrane Cylinder at pNom export=true name=FNom prio=1 dataSetName=cyl_dummy dataClassType=cyl dataClassName=$dataSetClassCyl$ unit='N' description='Nominal Force Membrane Cylinder at pNom': brakeCylinderTrailerA1_R.FNom [N]"; p153 "Maximum Cylinder Stroke export=true name=maxStroke prio=1 dataSetName=cyl_dummy dataClassType=cyl dataClassName=$dataSetClassCyl$ unit='m' description='Maximum Cylinder Stroke': brakeCylinderTrailerA1_R.maxStroke [m]"; p154 "Application Pressure Membrane Chamber (relative to pAtm) export=true name=pApp prio=1 dataSetName=cyl_dummy dataClassType=cyl dataClassName=$dataSetClassCyl$  unit='Pa' description='Application Pressure Membrane Chamber (relative to pAtm)': brakeCylinderTrailerA1_R.pApp [Pa]"; p155 "Nominal Pressure (relative to pAtm) export=true name=pNom prio=1 dataSetName=cyl_dummy dataClassType=cyl dataClassName=$dataSetClassCyl$ unit='Pa' description='Nominal Pressure (relative to pAtm)': brakeCylinderTrailerA1_R.pNom [Pa]"; p156 "Spring Brake Release Pressure (relative to pAtm) export=true name=pR_PB prio=1 dataSetName=cyl_dummy dataClassType=cyl dataClassName=$dataSetClassCyl$ unit='Pa' description='Spring Brake Release Pressure (relative to pAtm)': brakeCylinderTrailerA1_R.pR_PB [Pa]"; p157 "Spring Brake Release Stroke at pR_PB export=true name=xR_PB prio=1 dataSetName=cyl_dummy dataClassType=cyl dataClassName=$dataSetClassCyl$ unit='m' description='Spring Brake Release Stroke at pR_PB': brakeCylinderTrailerA1_R.xR_PB [m]"; p158 "Dimension of Parking Brake Spring Curve (max 10) export=true name=dxFSpring_Dim prio=1 dataSetName=cyl_dummy dataClassType=cyl dataClassName=$dataSetClassCyl$  unit='-' description='Dimension of Parking Brake Spring Curve (max 10)': brakeCylinderTrailerA2_R.dxFSpring_Dim [-]"; p159 "Dimension of Parking Brake Chamber Volume Curve (max 10) export=true name=dxVolPB_Dim prio=1 dataSetName=cyl_dummy dataClassType=cyl dataClassName=$dataSetClassCyl$  unit='-' description='Dimension of Parking Brake Chamber Volume Curve (max 10)': brakeCylinderTrailerA2_R.dxVolPB_Dim [-]"; p160 "Dimension of Service Brake Chamber Volume Curve (max 10) export=true name=dxVolSB_Dim prio=1 dataSetName=cyl_dummy dataClassType=cyl dataClassName=$dataSetClassCyl$  unit='-' description='Dimension of Service Brake Chamber Volume Curve (max 10)': brakeCylinderTrailerA2_R.dxVolSB_Dim [-]"; p161 "Nominal Force Membrane Cylinder at pNom export=true name=FNom prio=1 dataSetName=cyl_dummy dataClassType=cyl dataClassName=$dataSetClassCyl$ unit='N' description='Nominal Force Membrane Cylinder at pNom': brakeCylinderTrailerA2_R.FNom [N]"; p162 "Maximum Cylinder Stroke export=true name=maxStroke prio=1 dataSetName=cyl_dummy dataClassType=cyl dataClassName=$dataSetClassCyl$ unit='m' description='Maximum Cylinder Stroke': brakeCylinderTrailerA2_R.maxStroke [m]"; p163 "Application Pressure Membrane Chamber (relative to pAtm) export=true name=pApp prio=1 dataSetName=cyl_dummy dataClassType=cyl dataClassName=$dataSetClassCyl$  unit='Pa' description='Application Pressure Membrane Chamber (relative to pAtm)': brakeCylinderTrailerA2_R.pApp [Pa]"; p164 "Nominal Pressure (relative to pAtm) export=true name=pNom prio=1 dataSetName=cyl_dummy dataClassType=cyl dataClassName=$dataSetClassCyl$ unit='Pa' description='Nominal Pressure (relative to pAtm)': brakeCylinderTrailerA2_R.pNom [Pa]"; p165 "Spring Brake Release Pressure (relative to pAtm) export=true name=pR_PB prio=1 dataSetName=cyl_dummy dataClassType=cyl dataClassName=$dataSetClassCyl$ unit='Pa' description='Spring Brake Release Pressure (relative to pAtm)': brakeCylinderTrailerA2_R.pR_PB [Pa]"; p166 "Spring Brake Release Stroke at pR_PB export=true name=xR_PB prio=1 dataSetName=cyl_dummy dataClassType=cyl dataClassName=$dataSetClassCyl$ unit='m' description='Spring Brake Release Stroke at pR_PB': brakeCylinderTrailerA2_R.xR_PB [m]"; p167 "Dimension of Parking Brake Spring Curve (max 10) export=true name=dxFSpring_Dim prio=1 dataSetName=cyl_dummy dataClassType=cyl dataClassName=$dataSetClassCyl$  unit='-' description='Dimension of Parking Brake Spring Curve (max 10)': brakeCylinderTrailerA3_R.dxFSpring_Dim [-]"; p168 "Dimension of Parking Brake Chamber Volume Curve (max 10) export=true name=dxVolPB_Dim prio=1 dataSetName=cyl_dummy dataClassType=cyl dataClassName=$dataSetClassCyl$  unit='-' description='Dimension of Parking Brake Chamber Volume Curve (max 10)': brakeCylinderTrailerA3_R.dxVolPB_Dim [-]"; p169 "Dimension of Service Brake Chamber Volume Curve (max 10) export=true name=dxVolSB_Dim prio=1 dataSetName=cyl_dummy dataClassType=cyl dataClassName=$dataSetClassCyl$  unit='-' description='Dimension of Service Brake Chamber Volume Curve (max 10)': brakeCylinderTrailerA3_R.dxVolSB_Dim [-]"; p170 "Nominal Force Membrane Cylinder at pNom export=true name=FNom prio=1 dataSetName=cyl_dummy dataClassType=cyl dataClassName=$dataSetClassCyl$ unit='N' description='Nominal Force Membrane Cylinder at pNom': brakeCylinderTrailerA3_R.FNom [N]"; p171 "Maximum Cylinder Stroke export=true name=maxStroke prio=1 dataSetName=cyl_dummy dataClassType=cyl dataClassName=$dataSetClassCyl$ unit='m' description='Maximum Cylinder Stroke': brakeCylinderTrailerA3_R.maxStroke [m]"; p172 "Application Pressure Membrane Chamber (relative to pAtm) export=true name=pApp prio=1 dataSetName=cyl_dummy dataClassType=cyl dataClassName=$dataSetClassCyl$  unit='Pa' description='Application Pressure Membrane Chamber (relative to pAtm)': brakeCylinderTrailerA3_R.pApp [Pa]"; p173 "Nominal Pressure (relative to pAtm) export=true name=pNom prio=1 dataSetName=cyl_dummy dataClassType=cyl dataClassName=$dataSetClassCyl$ unit='Pa' description='Nominal Pressure (relative to pAtm)': brakeCylinderTrailerA3_R.pNom [Pa]"; p174 "Spring Brake Release Pressure (relative to pAtm) export=true name=pR_PB prio=1 dataSetName=cyl_dummy dataClassType=cyl dataClassName=$dataSetClassCyl$ unit='Pa' description='Spring Brake Release Pressure (relative to pAtm)': brakeCylinderTrailerA3_R.pR_PB [Pa]"; p175 "Spring Brake Release Stroke at pR_PB export=true name=xR_PB prio=1 dataSetName=cyl_dummy dataClassType=cyl dataClassName=$dataSetClassCyl$ unit='m' description='Spring Brake Release Stroke at pR_PB': brakeCylinderTrailerA3_R.xR_PB [m]"; p176 "Brake Type (Disc - 0, Drum - 1)  export=true name=brakeType prio=1 dataSetName=brk_dummy dataClassType=brk dataClassName=$dataSetClassBrk$ unit='-' description='Brake Type (Disc - 0, Drum - 1)': BrakeTrailerA1_R.brakeType [-]"; p177 "brake type dependent surface area [m^2] (C_TEM_A_NORM) export=true name=bt_A_norm prio=1 dataSetName=brk_dummy dataClassType=brk dataClassName=$dataSetClassBrk$  unit='m^2' description='brake type dependent surface area [m^2] (C_TEM_A_NORM)': BrakeTrailerA1_R.bt_A_norm [m²]"; p178 "brake pad friction area [m^2] export=true name=bt_A_pad prio=1 dataSetName=brk_dummy dataClassType=brk dataClassName=$dataSetClassBrk$  unit='m^2' description='brake pad friction area [m^2]': BrakeTrailerA1_R.bt_A_pad [m²]"; p179 "brake type dependent scaling for the heat loss due to convection at the cooling brake surface [-] (C_TEM_FAC_CONV_COOL) export=true name=bt_alpha_conv_fac_cool prio=1 dataSetName=brk_dummy dataClassType=brk dataClassName=$dataSetClassBrk$  unit='-' description='bbrake type dependent scaling for the heat loss due to convection at the cooling brake surface [-] (C_TEM_FAC_CONV_COOL)': BrakeTrailerA1_R.bt_alpha_conv_fac_cool [-]"; p180 "brake type dependent scaling for the heat loss due to convection at the friction brake surface [-] (C_TEM_FAC_CONV_FRIC) export=true name=bt_alpha_conv_fac_fric prio=1 dataSetName=brk_dummy dataClassType=brk dataClassName=$dataSetClassBrk$  unit='-' description='brake type dependent scaling for the heat loss due to convection at the friction brake surface [-] (C_TEM_FAC_CONV_FRIC)': BrakeTrailerA1_R.bt_alpha_conv_fac_fric [-]"; p181 "brake type dependent correction of heat loss due to conduction into the brake base [-] (C_TEM_CONDUCT_BASE) export=true name=bt_base_conduction_corr prio=1 dataSetName=brk_dummy dataClassType=brk dataClassName=$dataSetClassBrk$  unit='-' description='brake type dependent correction of heat loss due to conduction into the brake base [-] (C_TEM_CONDUCT_BASE)': BrakeTrailerA1_R.bt_base_conduction_corr [-]"; p182 "brake type dependent spatial discretization length [m] (C_TEM_DELTA_R) export=true name=bt_delta_r prio=1 dataSetName=brk_dummy dataClassType=brk dataClassName=$dataSetClassBrk$  unit='m' description='brake type dependent spatial discretization length [m] (C_TEM_DELTA_R)': BrakeTrailerA1_R.bt_delta_r [m]"; p183 "brake type dependent density correction [-] (C_TEM_DENSITY_CORR) export=true name=bt_density_correction prio=1 dataSetName=brk_dummy dataClassType=brk dataClassName=$dataSetClassBrk$  unit='-' description='brake type dependent density correction [-] (C_TEM_DENSITY_CORR)': BrakeTrailerA1_R.bt_density_correction [-]"; p184 "brake type dependent emission number [-] (C_TEM_EPSILON_BrakeType/C_TEM_EPSILON) export=true name=bt_epsilon_corr prio=1 dataSetName=brk_dummy dataClassType=brk dataClassName=$dataSetClassBrk$  unit='-' description='brake type dependent emission number [-] (C_TEM_EPSILON_BrakeType/C_TEM_EPSILON)': BrakeTrailerA1_R.bt_epsilon_corr [-]"; p185 "brake type dependent correction for cylindrical coordinates [-] (C_TEM_CYLINDER_CORR) export=true name=bt_rad_offset prio=1 dataSetName=brk_dummy dataClassType=brk dataClassName=$dataSetClassBrk$  unit='-' description='brake type dependent correction for cylindrical coordinates [-] (C_TEM_CYLINDER_CORR)': BrakeTrailerA1_R.bt_rad_offset [-]"; p186 "brake type dependent area correction for radiation [-] (C_TEM_RAD_AREA_CORR) export=true name=bt_radiation_area_corr prio=1 dataSetName=brk_dummy dataClassType=brk dataClassName=$dataSetClassBrk$  unit='-' description='brake type dependent area correction for radiation [-] (C_TEM_RAD_AREA_CORR)': BrakeTrailerA1_R.bt_radiation_area_corr [-]"; p187 "Consider Grinding Torque (0-false, 1-true) export=true name=considerTg prio=1 dataSetName=brk_dummy dataClassType=brk dataClassName=$dataSetClassBrk$  unit='-' description='Consider Grinding Torque (0-false, 1-true)': BrakeTrailerA1_R.considerTg [-]"; p188 "Brake Factor export=true name=Cs prio=1 dataSetName=brk_dummy dataClassType=brk dataClassName=$dataSetClassBrk$  unit='-' description='Brake Factor': BrakeTrailerA1_R.Cs [-]"; p189 "Efficiency export=true name=eta prio=1 dataSetName=brk_dummy dataClassType=brk dataClassName=$dataSetClassBrk$  unit='-' description='Efficiency': BrakeTrailerA1_R.eta [-]"; p190 "Dimension Temperature Correction Factor-Vector Length (max. 25) export=true name=fac_T_Dim prio=1 dataSetName=brk_dummy dataClassType=brk dataClassName=$dataSetClassBrk$  unit='-' description='Dimension Temperature Correction Factor-Vector Length (max. 25)': BrakeTrailerA1_R.fac_T_Dim [-]"; p191 "Dimension Velocity Correction Factor-Vector Length (max. 10) export=true name=fac_v_Dim prio=1 dataSetName=brk_dummy dataClassType=brk dataClassName=$dataSetClassBrk$  unit='-' description='Dimension Velocity Correction Factor-Vector Length (max. 10)': BrakeTrailerA1_R.fac_v_Dim [-]"; p192 "Dimension Fdx-Vector Length (max. 10) export=true name=Fdx_Dim prio=1 dataSetName=brk_dummy dataClassType=brk dataClassName=$dataSetClassBrk$  unit='-' description='Dimension Fdx-Vector Length (max. 10)': BrakeTrailerA1_R.Fdx_Dim [-]"; p193 "Gathering Factor Wear export=true name=Gwear prio=1 dataSetName=brk_dummy dataClassType=brk dataClassName=$dataSetClassBrk$  unit='-' description='Gathering Factor Wear': BrakeTrailerA1_R.Gwear [-]"; p194 "Dimension of i-dx-Vector Length (Transmission Ratio FBrake/FPiston) (max. 15) export=true name=i_Dim prio=1 dataSetName=brk_dummy dataClassType=brk dataClassName=$dataSetClassBrk$  unit='-' description='Dimension of i-dx-Vector Length (Transmission Ratio FBrake/FPiston) (max. 15)': BrakeTrailerA1_R.i_Dim [-]"; p195 "Effective Brake Radius export=true name=reff prio=1 dataSetName=brk_dummy dataClassType=brk dataClassName=$dataSetClassBrk$  unit='m' description='Effective Brake Radius': BrakeTrailerA1_R.reff [m]"; p196 "Initial Sum Brake Pad Thickness sPad_sum0 export=true name=sPad_sum0 prio=1 dataSetName=brk_dummy dataClassType=brk dataClassName=$dataSetClassBrk$  unit='m' description='Initial Sum Brake Pad Thickness sPad_sum0 [m]': BrakeTrailerA1_R.sPad_sum0 [m]"; p197 "Temperature calculation mode: 0 - constant temperature, 1 - variable temperature export=true name=useVarTempCalc prio=1 dataSetName=brk_dummy dataClassType=brk dataClassName=$dataSetClassBrk$  unit='-' description='Temperature calculation mode: 0 - constant temperature, 1 - variable temperature': BrakeTrailerA1_R.useVarTempCalc [-]"; p198 "Dimension Temperature Correction Factor-Vector Length (max. 20) export=true name=wearRate_T_Dim prio=1 dataSetName=brk_dummy dataClassType=brk dataClassName=$dataSetClassBrk$  unit='-' description='Dimension Temperature Correction Factor-Vector Length (max. 20)': BrakeTrailerA1_R.wearRate_T_Dim [-]"; p199 "Brake Type (Disc - 0, Drum - 1)  export=true name=brakeType prio=1 dataSetName=brk_dummy dataClassType=brk dataClassName=$dataSetClassBrk$ unit='-' description='Brake Type (Disc - 0, Drum - 1)': BrakeTrailerA2_R.brakeType [-]"; p200 "brake type dependent surface area [m^2] (C_TEM_A_NORM) export=true name=bt_A_norm prio=1 dataSetName=brk_dummy dataClassType=brk dataClassName=$dataSetClassBrk$  unit='m^2' description='brake type dependent surface area [m^2] (C_TEM_A_NORM)': BrakeTrailerA2_R.bt_A_norm [m²]"; p201 "brake pad friction area [m^2] export=true name=bt_A_pad prio=1 dataSetName=brk_dummy dataClassType=brk dataClassName=$dataSetClassBrk$  unit='m^2' description='brake pad friction area [m^2]': BrakeTrailerA2_R.bt_A_pad [m²]"; p202 "brake type dependent scaling for the heat loss due to convection at the cooling brake surface [-] (C_TEM_FAC_CONV_COOL) export=true name=bt_alpha_conv_fac_cool prio=1 dataSetName=brk_dummy dataClassType=brk dataClassName=$dataSetClassBrk$  unit='-' description='bbrake type dependent scaling for the heat loss due to convection at the cooling brake surface [-] (C_TEM_FAC_CONV_COOL)': BrakeTrailerA2_R.bt_alpha_conv_fac_cool [-]"; p203 "brake type dependent scaling for the heat loss due to convection at the friction brake surface [-] (C_TEM_FAC_CONV_FRIC) export=true name=bt_alpha_conv_fac_fric prio=1 dataSetName=brk_dummy dataClassType=brk dataClassName=$dataSetClassBrk$  unit='-' description='brake type dependent scaling for the heat loss due to convection at the friction brake surface [-] (C_TEM_FAC_CONV_FRIC)': BrakeTrailerA2_R.bt_alpha_conv_fac_fric [-]"; p204 "brake type dependent correction of heat loss due to conduction into the brake base [-] (C_TEM_CONDUCT_BASE) export=true name=bt_base_conduction_corr prio=1 dataSetName=brk_dummy dataClassType=brk dataClassName=$dataSetClassBrk$  unit='-' description='brake type dependent correction of heat loss due to conduction into the brake base [-] (C_TEM_CONDUCT_BASE)': BrakeTrailerA2_R.bt_base_conduction_corr [-]"; p205 "brake type dependent spatial discretization length [m] (C_TEM_DELTA_R) export=true name=bt_delta_r prio=1 dataSetName=brk_dummy dataClassType=brk dataClassName=$dataSetClassBrk$  unit='m' description='brake type dependent spatial discretization length [m] (C_TEM_DELTA_R)': BrakeTrailerA2_R.bt_delta_r [m]"; p206 "brake type dependent density correction [-] (C_TEM_DENSITY_CORR) export=true name=bt_density_correction prio=1 dataSetName=brk_dummy dataClassType=brk dataClassName=$dataSetClassBrk$  unit='-' description='brake type dependent density correction [-] (C_TEM_DENSITY_CORR)': BrakeTrailerA2_R.bt_density_correction [-]"; p207 "brake type dependent emission number [-] (C_TEM_EPSILON_BrakeType/C_TEM_EPSILON) export=true name=bt_epsilon_corr prio=1 dataSetName=brk_dummy dataClassType=brk dataClassName=$dataSetClassBrk$  unit='-' description='brake type dependent emission number [-] (C_TEM_EPSILON_BrakeType/C_TEM_EPSILON)': BrakeTrailerA2_R.bt_epsilon_corr [-]"; p208 "brake type dependent correction for cylindrical coordinates [-] (C_TEM_CYLINDER_CORR) export=true name=bt_rad_offset prio=1 dataSetName=brk_dummy dataClassType=brk dataClassName=$dataSetClassBrk$  unit='-' description='brake type dependent correction for cylindrical coordinates [-] (C_TEM_CYLINDER_CORR)': BrakeTrailerA2_R.bt_rad_offset [-]"; p209 "brake type dependent area correction for radiation [-] (C_TEM_RAD_AREA_CORR) export=true name=bt_radiation_area_corr prio=1 dataSetName=brk_dummy dataClassType=brk dataClassName=$dataSetClassBrk$  unit='-' description='brake type dependent area correction for radiation [-] (C_TEM_RAD_AREA_CORR)': BrakeTrailerA2_R.bt_radiation_area_corr [-]"; p210 "Consider Grinding Torque (0-false, 1-true) export=true name=considerTg prio=1 dataSetName=brk_dummy dataClassType=brk dataClassName=$dataSetClassBrk$  unit='-' description='Consider Grinding Torque (0-false, 1-true)': BrakeTrailerA2_R.considerTg [-]"; p211 "Brake Factor export=true name=Cs prio=1 dataSetName=brk_dummy dataClassType=brk dataClassName=$dataSetClassBrk$  unit='-' description='Brake Factor': BrakeTrailerA2_R.Cs [-]"; p212 "Efficiency export=true name=eta prio=1 dataSetName=brk_dummy dataClassType=brk dataClassName=$dataSetClassBrk$  unit='-' description='Efficiency': BrakeTrailerA2_R.eta [-]"; p213 "Dimension Temperature Correction Factor-Vector Length (max. 25) export=true name=fac_T_Dim prio=1 dataSetName=brk_dummy dataClassType=brk dataClassName=$dataSetClassBrk$  unit='-' description='Dimension Temperature Correction Factor-Vector Length (max. 25)': BrakeTrailerA2_R.fac_T_Dim [-]"; p214 "Dimension Velocity Correction Factor-Vector Length (max. 10) export=true name=fac_v_Dim prio=1 dataSetName=brk_dummy dataClassType=brk dataClassName=$dataSetClassBrk$  unit='-' description='Dimension Velocity Correction Factor-Vector Length (max. 10)': BrakeTrailerA2_R.fac_v_Dim [-]"; p215 "Dimension Fdx-Vector Length (max. 10) export=true name=Fdx_Dim prio=1 dataSetName=brk_dummy dataClassType=brk dataClassName=$dataSetClassBrk$  unit='-' description='Dimension Fdx-Vector Length (max. 10)': BrakeTrailerA2_R.Fdx_Dim [-]"; p216 "Gathering Factor Wear export=true name=Gwear prio=1 dataSetName=brk_dummy dataClassType=brk dataClassName=$dataSetClassBrk$  unit='-' description='Gathering Factor Wear': BrakeTrailerA2_R.Gwear [-]"; p217 "Dimension of i-dx-Vector Length (Transmission Ratio FBrake/FPiston) (max. 15) export=true name=i_Dim prio=1 dataSetName=brk_dummy dataClassType=brk dataClassName=$dataSetClassBrk$  unit='-' description='Dimension of i-dx-Vector Length (Transmission Ratio FBrake/FPiston) (max. 15)': BrakeTrailerA2_R.i_Dim [-]"; p218 "Effective Brake Radius export=true name=reff prio=1 dataSetName=brk_dummy dataClassType=brk dataClassName=$dataSetClassBrk$  unit='m' description='Effective Brake Radius': BrakeTrailerA2_R.reff [m]"; p219 "Initial Sum Brake Pad Thickness sPad_sum0 export=true name=sPad_sum0 prio=1 dataSetName=brk_dummy dataClassType=brk dataClassName=$dataSetClassBrk$  unit='m' description='Initial Sum Brake Pad Thickness sPad_sum0 [m]': BrakeTrailerA2_R.sPad_sum0 [m]"; p220 "Temperature calculation mode: 0 - constant temperature, 1 - variable temperature export=true name=useVarTempCalc prio=1 dataSetName=brk_dummy dataClassType=brk dataClassName=$dataSetClassBrk$  unit='-' description='Temperature calculation mode: 0 - constant temperature, 1 - variable temperature': BrakeTrailerA2_R.useVarTempCalc [-]"; p221 "Dimension Temperature Correction Factor-Vector Length (max. 20) export=true name=wearRate_T_Dim prio=1 dataSetName=brk_dummy dataClassType=brk dataClassName=$dataSetClassBrk$  unit='-' description='Dimension Temperature Correction Factor-Vector Length (max. 20)': BrakeTrailerA2_R.wearRate_T_Dim [-]"; p222 "Brake Type (Disc - 0, Drum - 1)  export=true name=brakeType prio=1 dataSetName=brk_dummy dataClassType=brk dataClassName=$dataSetClassBrk$ unit='-' description='Brake Type (Disc - 0, Drum - 1)': BrakeTrailerA3_R.brakeType [-]"; p223 "brake type dependent surface area [m^2] (C_TEM_A_NORM) export=true name=bt_A_norm prio=1 dataSetName=brk_dummy dataClassType=brk dataClassName=$dataSetClassBrk$  unit='m^2' description='brake type dependent surface area [m^2] (C_TEM_A_NORM)': BrakeTrailerA3_R.bt_A_norm [m²]"; p224 "brake pad friction area [m^2] export=true name=bt_A_pad prio=1 dataSetName=brk_dummy dataClassType=brk dataClassName=$dataSetClassBrk$  unit='m^2' description='brake pad friction area [m^2]': BrakeTrailerA3_R.bt_A_pad [m²]"; p225 "brake type dependent scaling for the heat loss due to convection at the cooling brake surface [-] (C_TEM_FAC_CONV_COOL) export=true name=bt_alpha_conv_fac_cool prio=1 dataSetName=brk_dummy dataClassType=brk dataClassName=$dataSetClassBrk$  unit='-' description='bbrake type dependent scaling for the heat loss due to convection at the cooling brake surface [-] (C_TEM_FAC_CONV_COOL)': BrakeTrailerA3_R.bt_alpha_conv_fac_cool [-]"; p226 "brake type dependent scaling for the heat loss due to convection at the friction brake surface [-] (C_TEM_FAC_CONV_FRIC) export=true name=bt_alpha_conv_fac_fric prio=1 dataSetName=brk_dummy dataClassType=brk dataClassName=$dataSetClassBrk$  unit='-' description='brake type dependent scaling for the heat loss due to convection at the friction brake surface [-] (C_TEM_FAC_CONV_FRIC)': BrakeTrailerA3_R.bt_alpha_conv_fac_fric [-]"; p227 "brake type dependent correction of heat loss due to conduction into the brake base [-] (C_TEM_CONDUCT_BASE) export=true name=bt_base_conduction_corr prio=1 dataSetName=brk_dummy dataClassType=brk dataClassName=$dataSetClassBrk$  unit='-' description='brake type dependent correction of heat loss due to conduction into the brake base [-] (C_TEM_CONDUCT_BASE)': BrakeTrailerA3_R.bt_base_conduction_corr [-]"; p228 "brake type dependent spatial discretization length [m] (C_TEM_DELTA_R) export=true name=bt_delta_r prio=1 dataSetName=brk_dummy dataClassType=brk dataClassName=$dataSetClassBrk$  unit='m' description='brake type dependent spatial discretization length [m] (C_TEM_DELTA_R)': BrakeTrailerA3_R.bt_delta_r [m]"; p229 "brake type dependent density correction [-] (C_TEM_DENSITY_CORR) export=true name=bt_density_correction prio=1 dataSetName=brk_dummy dataClassType=brk dataClassName=$dataSetClassBrk$  unit='-' description='brake type dependent density correction [-] (C_TEM_DENSITY_CORR)': BrakeTrailerA3_R.bt_density_correction [-]"; p230 "brake type dependent emission number [-] (C_TEM_EPSILON_BrakeType/C_TEM_EPSILON) export=true name=bt_epsilon_corr prio=1 dataSetName=brk_dummy dataClassType=brk dataClassName=$dataSetClassBrk$  unit='-' description='brake type dependent emission number [-] (C_TEM_EPSILON_BrakeType/C_TEM_EPSILON)': BrakeTrailerA3_R.bt_epsilon_corr [-]"; p231 "brake type dependent correction for cylindrical coordinates [-] (C_TEM_CYLINDER_CORR) export=true name=bt_rad_offset prio=1 dataSetName=brk_dummy dataClassType=brk dataClassName=$dataSetClassBrk$  unit='-' description='brake type dependent correction for cylindrical coordinates [-] (C_TEM_CYLINDER_CORR)': BrakeTrailerA3_R.bt_rad_offset [-]"; p232 "brake type dependent area correction for radiation [-] (C_TEM_RAD_AREA_CORR) export=true name=bt_radiation_area_corr prio=1 dataSetName=brk_dummy dataClassType=brk dataClassName=$dataSetClassBrk$  unit='-' description='brake type dependent area correction for radiation [-] (C_TEM_RAD_AREA_CORR)': BrakeTrailerA3_R.bt_radiation_area_corr [-]"; p233 "Consider Grinding Torque (0-false, 1-true) export=true name=considerTg prio=1 dataSetName=brk_dummy dataClassType=brk dataClassName=$dataSetClassBrk$  unit='-' description='Consider Grinding Torque (0-false, 1-true)': BrakeTrailerA3_R.considerTg [-]"; p234 "Brake Factor export=true name=Cs prio=1 dataSetName=brk_dummy dataClassType=brk dataClassName=$dataSetClassBrk$  unit='-' description='Brake Factor': BrakeTrailerA3_R.Cs [-]"; p235 "Efficiency export=true name=eta prio=1 dataSetName=brk_dummy dataClassType=brk dataClassName=$dataSetClassBrk$  unit='-' description='Efficiency': BrakeTrailerA3_R.eta [-]"; p236 "Dimension Temperature Correction Factor-Vector Length (max. 25) export=true name=fac_T_Dim prio=1 dataSetName=brk_dummy dataClassType=brk dataClassName=$dataSetClassBrk$  unit='-' description='Dimension Temperature Correction Factor-Vector Length (max. 25)': BrakeTrailerA3_R.fac_T_Dim [-]"; p237 "Dimension Velocity Correction Factor-Vector Length (max. 10) export=true name=fac_v_Dim prio=1 dataSetName=brk_dummy dataClassType=brk dataClassName=$dataSetClassBrk$  unit='-' description='Dimension Velocity Correction Factor-Vector Length (max. 10)': BrakeTrailerA3_R.fac_v_Dim [-]"; p238 "Dimension Fdx-Vector Length (max. 10) export=true name=Fdx_Dim prio=1 dataSetName=brk_dummy dataClassType=brk dataClassName=$dataSetClassBrk$  unit='-' description='Dimension Fdx-Vector Length (max. 10)': BrakeTrailerA3_R.Fdx_Dim [-]"; p239 "Gathering Factor Wear export=true name=Gwear prio=1 dataSetName=brk_dummy dataClassType=brk dataClassName=$dataSetClassBrk$  unit='-' description='Gathering Factor Wear': BrakeTrailerA3_R.Gwear [-]"; p240 "Dimension of i-dx-Vector Length (Transmission Ratio FBrake/FPiston) (max. 15) export=true name=i_Dim prio=1 dataSetName=brk_dummy dataClassType=brk dataClassName=$dataSetClassBrk$  unit='-' description='Dimension of i-dx-Vector Length (Transmission Ratio FBrake/FPiston) (max. 15)': BrakeTrailerA3_R.i_Dim [-]"; p241 "Effective Brake Radius export=true name=reff prio=1 dataSetName=brk_dummy dataClassType=brk dataClassName=$dataSetClassBrk$  unit='m' description='Effective Brake Radius': BrakeTrailerA3_R.reff [m]"; p242 "Initial Sum Brake Pad Thickness sPad_sum0 export=true name=sPad_sum0 prio=1 dataSetName=brk_dummy dataClassType=brk dataClassName=$dataSetClassBrk$  unit='m' description='Initial Sum Brake Pad Thickness sPad_sum0 [m]': BrakeTrailerA3_R.sPad_sum0 [m]"; p243 "Temperature calculation mode: 0 - constant temperature, 1 - variable temperature export=true name=useVarTempCalc prio=1 dataSetName=brk_dummy dataClassType=brk dataClassName=$dataSetClassBrk$  unit='-' description='Temperature calculation mode: 0 - constant temperature, 1 - variable temperature': BrakeTrailerA3_R.useVarTempCalc [-]"; p244 "Dimension Temperature Correction Factor-Vector Length (max. 20) export=true name=wearRate_T_Dim prio=1 dataSetName=brk_dummy dataClassType=brk dataClassName=$dataSetClassBrk$  unit='-' description='Dimension Temperature Correction Factor-Vector Length (max. 20)': BrakeTrailerA3_R.wearRate_T_Dim [-]"; p245 "Time Constant (PT1) Pipe AM Front - ABS Valve Front Left in [s] export=true name=T_pipe_AM_ABSValve_FL prio=1 dataSetName=circ_dummy dataClassType=circ dataClassName=circ unit='-' description='Time Constant (PT1) Pipe AM Front - ABS Valve Front Left in [s]': brkCircuit.T_pipe_AM_ABSValve_FL [s]"; p246 "Time Constant (PT1) Pipe AM Front - ABS Valve Front Right in [s] export=true name=T_pipe_AM_ABSValve_FR prio=1 dataSetName=circ_dummy dataClassType=circ dataClassName=circ unit='-' description='Time Constant (PT1) Pipe AM Front - ABS Valve Front Right in [s]': brkCircuit.T_pipe_AM_ABSValve_FR [s]"; p247 "Time Constant (PT1) Pipe AM Add - Brake Chamber Add Left in [s] export=true name=T_pipe_AM_BC_AL prio=1 dataSetName=circ_dummy dataClassType=circ dataClassName=circ unit='-' description='Time Constant (PT1) Pipe AM Add - Brake Chamber Add Left in [s]': brkCircuit.T_pipe_AM_BC_AL [s]"; p248 "Time Constant (PT1) Pipe AM Add - Brake Chamber Add Right in [s] export=true name=T_pipe_AM_BC_AR prio=1 dataSetName=circ_dummy dataClassType=circ dataClassName=circ unit='-' description='Time Constant (PT1) Pipe AM Add - Brake Chamber Add Right in [s]': brkCircuit.T_pipe_AM_BC_AR [s]"; p249 "Time Constant (PT1) Pipe AM Rear - Brake Chamber Rear Left in [s] export=true name=T_pipe_AM_BC_RL prio=1 dataSetName=circ_dummy dataClassType=circ dataClassName=circ unit='-' description='Time Constant (PT1) Pipe AM Rear - Brake Chamber Rear Left in [s]': brkCircuit.T_pipe_AM_BC_RL [s]"; p250 "Time Constant (PT1) Pipe AM Rear - Brake Chamber Rear Right in [s] export=true name=T_pipe_AM_BC_RR prio=1 dataSetName=circ_dummy dataClassType=circ dataClassName=circ unit='-' description='Time Constant (PT1) Pipe AM Rear - Brake Chamber Rear Right in [s]': brkCircuit.T_pipe_AM_BC_RR [s]"; p251 "Trailer ABS Config (0 - none, 1- ABS, 2 - EBS (incl. ABS)), used in pneAux export=true name=flagTrailerABS prio=1 dataSetName=circTrlr_dummy dataClassType=circTrlr dataClassName=circTrlr unit='-' description='Trailer ABS Config (0 - none, 1- ABS, 2 - EBS (incl. ABS))': brkCircuitTrlr.flagTrailerABS [-]"; p252 "Time Constant (PT1) Pipe TCV - Relais Valve Trailer Front Axle in [s] export=true name=T_pipe_Trailer_RV_Front prio=1 dataSetName=circTrlr_dummy dataClassType=circTrlr dataClassName=circTrlr unit='-' description='Time Constant (PT1) Pipe TCV - Relais Valve Trailer Front Axle in [s]': brkCircuitTrlr.T_pipe_Trailer_RV_Front [s]"; p253 "Time Constant (PT1) Pipe Relais Valve Trailer Front to Rear Axle in [s] export=true name=T_pipe_Trailer_RV_Front_Rear prio=1 dataSetName=circTrlr_dummy dataClassType=circTrlr dataClassName=circTrlr unit='-' description='Time Constant (PT1) Pipe Relais Valve Trailer Front to Rear Axle in [s]': brkCircuitTrlr.T_pipe_Trailer_RV_Front_Rear [s]"; p254 "Volume Tank Trailer [dm^3] export=true name=VTrailer prio=1 dataSetName=circTrlr_dummy dataClassType=circTrlr dataClassName=circTrlr unit='dm^3' description='Volume Tank Trailer [dm^3]': brkCircuitTrlr.VTrailer [-]"; p255 "Air Compressor Overflow Pressure [bar] export=true name=pACoverflow prio=1 dataSetName=com_dummy dataClassType=com dataClassName=com unit='bar' description='Air Compressor Overflow Pressure [bar]': compressor.pACoverflow [-]"; p256 "Air Consumption Door Closing [l] export=true name=Drs_dVClose prio=1 dataSetName=auxil_dummy dataClassType=auxil dataClassName=auxil unit='l' description='Air Consumption Door Closing [l]': doors.Drs_dVClose [-]"; p257 "Air Consumption Door Opening [l] export=true name=Drs_dVOpen prio=1 dataSetName=auxil_dummy dataClassType=auxil dataClassName=auxil unit='l' description='Air Consumption Door Opening [l]': doors.Drs_dVOpen [-]"; p258 "Measurement Pressure (absolute) [bar] export=true name=Drs_pMeas prio=1 dataSetName=auxil_dummy dataClassType=auxil dataClassName=auxil unit='bar' description='Measurement Pressure (absolute) [bar]': doors.Drs_pMeas [-]"; p259 "Door Closing Time [s] export=true name=Drs_tClose prio=1 dataSetName=auxil_dummy dataClassType=auxil dataClassName=auxil unit='s' description='Door Closing Time [s]': doors.Drs_tClose [s]"; p260 "Door Opening Time [s] export=true name=Drs_tOpen prio=1 dataSetName=auxil_dummy dataClassType=auxil dataClassName=auxil unit='s' description='Door Opening Time [s]': doors.Drs_tOpen [s]"; p261 "ebs_AdditionalAxle_left_pDmd (init) export=true name=ebs_AdditionalAxle_left_pDmd prio=1 dataSetName=std dataClassType=initIO dataClassName=initIO unit='-' description='ebs_AdditionalAxle_left_pDmd': IO_PNE_Generic.ebs_AdditionalAxle_left_pDmd_0 [-]"; p262 "ebs_AdditionalAxle_left_setABS (init) export=true name=ebs_AdditionalAxle_left_setABS prio=1 dataSetName=std dataClassType=initIO dataClassName=initIO unit='-' description='ebs_AdditionalAxle_left_setABS': IO_PNE_Generic.ebs_AdditionalAxle_left_setABS_0 [-]"; p263 "ebs_AdditionalAxle_right_pDmd (init) export=true name=ebs_AdditionalAxle_right_pDmd prio=1 dataSetName=std dataClassType=initIO dataClassName=initIO unit='-' description='ebs_AdditionalAxle_right_pDmd': IO_PNE_Generic.ebs_AdditionalAxle_right_pDmd_0 [-]"; p264 "ebs_AdditionalAxle_right_setABS (init) export=true name=ebs_AdditionalAxle_right_setABS prio=1 dataSetName=std dataClassType=initIO dataClassName=initIO unit='-' description='ebs_AdditionalAxle_right_setABS': IO_PNE_Generic.ebs_AdditionalAxle_right_setABS_0 [-]"; p265 "ebs_ESCsens_y_acceleration (init) export=true name=ebs_ESCsens_y_acceleration prio=1 dataSetName=std dataClassType=initIO dataClassName=initIO unit=mbar description='env_pressure': IO_PNE_Generic.ebs_ESCsens_y_acceleration_0 [-]"; p266 "ebs_FrontAxle_left_pDmd (init) export=true name=ebs_FrontAxle_left_pDmd prio=1 dataSetName=std dataClassType=initIO dataClassName=initIO unit='-' description='ebs_FrontAxle_left_pDmd': IO_PNE_Generic.ebs_FrontAxle_left_pDmd_0 [-]"; p267 "ebs_FrontAxle_left_setABS (init) export=true name=ebs_FrontAxle_left_setABS prio=1 dataSetName=std dataClassType=initIO dataClassName=initIO unit='-' description='ebs_FrontAxle_left_setABS': IO_PNE_Generic.ebs_FrontAxle_left_setABS_0 [-]"; p268 "ebs_FrontAxle_right_pDmd (init) export=true name=ebs_FrontAxle_right_pDmd prio=1 dataSetName=std dataClassType=initIO dataClassName=initIO unit='-' description='ebs_FrontAxle_right_pDmd': IO_PNE_Generic.ebs_FrontAxle_right_pDmd_0 [-]"; p269 "ebs_FrontAxle_right_setABS (init) export=true name=ebs_FrontAxle_right_setABS prio=1 dataSetName=std dataClassType=initIO dataClassName=initIO unit='-' description='ebs_FrontAxle_right_setABS': IO_PNE_Generic.ebs_FrontAxle_right_setABS_0 [-]"; p270 "ebs_RearAxle_left_pDmd (init) export=true name=ebs_RearAxle_left_pDmd prio=1 dataSetName=std dataClassType=initIO dataClassName=initIO unit='-' description='ebs_RearAxle_left_pDmd': IO_PNE_Generic.ebs_RearAxle_left_pDmd_0 [-]"; p271 "ebs_RearAxle_left_setABS (init) export=true name=ebs_RearAxle_left_setABS prio=1 dataSetName=std dataClassType=initIO dataClassName=initIO unit='-' description='ebs_RearAxle_left_setABS': IO_PNE_Generic.ebs_RearAxle_left_setABS_0 [-]"; p272 "ebs_RearAxle_right_pDmd (init) export=true name=ebs_RearAxle_right_pDmd prio=1 dataSetName=std dataClassType=initIO dataClassName=initIO unit='-' description='ebs_RearAxle_right_pDmd': IO_PNE_Generic.ebs_RearAxle_right_pDmd_0 [-]"; p273 "ebs_RearAxle_right_setABS (init) export=true name=ebs_RearAxle_right_setABS prio=1 dataSetName=std dataClassType=initIO dataClassName=initIO unit='-' description='ebs_RearAxle_right_setABS': IO_PNE_Generic.ebs_RearAxle_right_setABS_0 [-]"; p274 "ebs_sBSP_stABSInValve_Addl_Left (init) export=true name=ebs_sBSP_stABSInValve_Addl_Left prio=1 dataSetName=std dataClassType=initIO dataClassName=initIO unit='-' description='ebs_sBSP_stABSInValve_Addl_Left': IO_PNE_Generic.ebs_sBSP_stABSInValve_Addl_Left_0 [-]"; p275 "ebs_sBSP_stABSInValve_Addl_Right (init) export=true name=ebs_sBSP_stABSInValve_Addl_Right prio=1 dataSetName=std dataClassType=initIO dataClassName=initIO unit='-' description='ebs_sBSP_stABSInValve_Addl_Right': IO_PNE_Generic.ebs_sBSP_stABSInValve_Addl_Right_0 [-]"; p276 "ebs_sBSP_stABSInValve_Front_Left (init) export=true name=ebs_sBSP_stABSInValve_Front_Left prio=1 dataSetName=std dataClassType=initIO dataClassName=initIO unit='-' description='ebs_sBSP_stABSInValve_Front_Left': IO_PNE_Generic.ebs_sBSP_stABSInValve_Front_Left_0 [-]"; p277 "ebs_sBSP_stABSInValve_Front_Right (init) export=true name=ebs_sBSP_stABSInValve_Front_Right prio=1 dataSetName=std dataClassType=initIO dataClassName=initIO unit='-' description='ebs_sBSP_stABSInValve_Front_Right': IO_PNE_Generic.ebs_sBSP_stABSInValve_Front_Right_0 [-]"; p278 "ebs_sBSP_stABSInValve_RCMax_Front,   export=true name=ebs_sBSP_stABSInValve_RCMax_Front prio=1 dataSetName=std dataClassType=initIO dataClassName=initIO unit='-' description=' ': IO_PNE_Generic.ebs_sBSP_stABSInValve_RCMax_Front_0 [-]"; p279 "ebs_sBSP_stABSInValve_RCMax_Rear,   export=true name=ebs_sBSP_stABSInValve_RCMax_Rear prio=1 dataSetName=std dataClassType=initIO dataClassName=initIO unit='-' description=' ': IO_PNE_Generic.ebs_sBSP_stABSInValve_RCMax_Rear_0 [-]"; p280 "ebs_sBSP_stABSInValve_Rear_Left (init) export=true name=ebs_sBSP_stABSInValve_Rear_Left prio=1 dataSetName=std dataClassType=initIO dataClassName=initIO unit='-' description='ebs_sBSP_stABSInValve_Rear_Left': IO_PNE_Generic.ebs_sBSP_stABSInValve_Rear_Left_0 [-]"; p281 "ebs_sBSP_stABSInValve_Rear_Right (init) export=true name=ebs_sBSP_stABSInValve_Rear_Right prio=1 dataSetName=std dataClassType=initIO dataClassName=initIO unit='-' description='ebs_sBSP_stABSInValve_Rear_Right': IO_PNE_Generic.ebs_sBSP_stABSInValve_Rear_Right_0 [-]"; p282 "ebs_sBSP_stABSOutValve_Addl_Left (init) export=true name=ebs_sBSP_stABSOutValve_Addl_Left prio=1 dataSetName=std dataClassType=initIO dataClassName=initIO unit='-' description='ebs_sBSP_stABSOutValve_Addl_Left': IO_PNE_Generic.ebs_sBSP_stABSOutValve_Addl_Left_0 [-]"; p283 "ebs_sBSP_stABSOutValve_Addl_Right (init) export=true name=ebs_sBSP_stABSOutValve_Addl_Right prio=1 dataSetName=std dataClassType=initIO dataClassName=initIO unit='-' description='ebs_sBSP_stABSOutValve_Addl_Right': IO_PNE_Generic.ebs_sBSP_stABSOutValve_Addl_Right_0 [-]"; p284 "ebs_sBSP_stABSOutValve_Front_Left (init) export=true name=ebs_sBSP_stABSOutValve_Front_Left prio=1 dataSetName=std dataClassType=initIO dataClassName=initIO unit='-' description='ebs_sBSP_stABSOutValve_Front_Left': IO_PNE_Generic.ebs_sBSP_stABSOutValve_Front_Left_0 [-]"; p285 "ebs_sBSP_stABSOutValve_Front_Right (init) export=true name=ebs_sBSP_stABSOutValve_Front_Right prio=1 dataSetName=std dataClassType=initIO dataClassName=initIO unit='-' description='ebs_sBSP_stABSOutValve_Front_Right': IO_PNE_Generic.ebs_sBSP_stABSOutValve_Front_Right_0 [-]"; p286 "ebs_sBSP_stABSOutValve_RCMax_Front,   export=true name=ebs_sBSP_stABSOutValve_RCMax_Front prio=1 dataSetName=std dataClassType=initIO dataClassName=initIO unit='-' description=' ': IO_PNE_Generic.ebs_sBSP_stABSOutValve_RCMax_Front_0 [-]"; p287 "ebs_sBSP_stABSOutValve_RCMax_Rear,   export=true name=ebs_sBSP_stABSOutValve_RCMax_Rear prio=1 dataSetName=std dataClassType=initIO dataClassName=initIO unit='-' description=' ': IO_PNE_Generic.ebs_sBSP_stABSOutValve_RCMax_Rear_0 [-]"; p288 "ebs_sBSP_stABSOutValve_Rear_Left (init) export=true name=ebs_sBSP_stABSOutValve_Rear_Left prio=1 dataSetName=std dataClassType=initIO dataClassName=initIO unit='-' description='ebs_sBSP_stABSOutValve_Rear_Left': IO_PNE_Generic.ebs_sBSP_stABSOutValve_Rear_Left_0 [-]"; p289 "ebs_sBSP_stABSOutValve_Rear_Right (init) export=true name=ebs_sBSP_stABSOutValve_Rear_Right prio=1 dataSetName=std dataClassType=initIO dataClassName=initIO unit='-' description='ebs_sBSP_stABSOutValve_Rear_Right': IO_PNE_Generic.ebs_sBSP_stABSOutValve_Rear_Right_0 [-]"; p290 "ebs_sBSP_stAPCVBuValve (init) export=true name=ebs_sBSP_stAPCVBuValve prio=1 dataSetName=std dataClassType=initIO dataClassName=initIO unit='-' description='ebs_sBSP_stAPCVBuValve': IO_PNE_Generic.ebs_sBSP_stAPCVBuValve_0 [-]"; p291 "ebs_sBSP_stAPCVInValve (init) export=true name=ebs_sBSP_stAPCVInValve prio=1 dataSetName=std dataClassType=initIO dataClassName=initIO unit='-' description='ebs_sBSP_stAPCVInValve': IO_PNE_Generic.ebs_sBSP_stAPCVInValve_0 [-]"; p292 "ebs_sBSP_stAPCVOutValve (init) export=true name=ebs_sBSP_stAPCVOutValve prio=1 dataSetName=std dataClassType=initIO dataClassName=initIO unit='-' description='ebs_sBSP_stAPCVOutValve': IO_PNE_Generic.ebs_sBSP_stAPCVOutValve_0 [-]"; p293 "ebs_sBSP_stAtcCutOffValve (init) export=true name=ebs_sBSP_stAtcCutOffValve prio=1 dataSetName=std dataClassType=initIO dataClassName=initIO unit='-' description='ebs_sBSP_stAtcCutOffValve': IO_PNE_Generic.ebs_sBSP_stAtcCutOffValve_0 [-]"; p294 "ebs_sBSP_stAxmoBuValve (init) export=true name=ebs_sBSP_stAxmoBuValve prio=1 dataSetName=std dataClassType=initIO dataClassName=initIO unit='-' description='ebs_sBSP_stAxmoBuValve': IO_PNE_Generic.ebs_sBSP_stAxmoBuValve_0 [-]"; p295 "ebs_sBSP_stAxmoInValve_Rear_Left (init) export=true name=ebs_sBSP_stAxmoInValve_Rear_Left prio=1 dataSetName=std dataClassType=initIO dataClassName=initIO unit='-' description='ebs_sBSP_stAxmoInValve_Rear_Left': IO_PNE_Generic.ebs_sBSP_stAxmoInValve_Rear_Left_0 [-]"; p296 "ebs_sBSP_stAxmoInValve_Rear_Right (init) export=true name=ebs_sBSP_stAxmoInValve_Rear_Right prio=1 dataSetName=std dataClassType=initIO dataClassName=initIO unit='-' description='ebs_sBSP_stAxmoInValve_Rear_Right': IO_PNE_Generic.ebs_sBSP_stAxmoInValve_Rear_Right_0 [-]"; p297 "ebs_sBSP_stAxmoOutValve_Rear_Left (init) export=true name=ebs_sBSP_stAxmoOutValve_Rear_Left prio=1 dataSetName=std dataClassType=initIO dataClassName=initIO unit='-' description='ebs_sBSP_stAxmoOutValve_Rear_Left': IO_PNE_Generic.ebs_sBSP_stAxmoOutValve_Rear_Left_0 [-]"; p298 "ebs_sBSP_stAxmoOutValve_Rear_Right (init) export=true name=ebs_sBSP_stAxmoOutValve_Rear_Right prio=1 dataSetName=std dataClassType=initIO dataClassName=initIO unit='-' description='ebs_sBSP_stAxmoOutValve_Rear_Right': IO_PNE_Generic.ebs_sBSP_stAxmoOutValve_Rear_Right_0 [-]"; p299 "ebs_sBSP_stCMaxBuValve (init) export=true name=ebs_sBSP_stCMaxBuValve prio=1 dataSetName=std dataClassType=initIO dataClassName=initIO unit='-' description='ebs_sBSP_stCMaxBuValve': IO_PNE_Generic.ebs_sBSP_stCMaxBuValve_0 [-]"; p300 "ebs_sBSP_stCMaxInValve_Rear_Left (init) export=true name=ebs_sBSP_stCMaxInValve_Rear_Left prio=1 dataSetName=std dataClassType=initIO dataClassName=initIO unit='-' description='ebs_sBSP_stCMaxInValve_Rear_Left': IO_PNE_Generic.ebs_sBSP_stCMaxInValve_Rear_Left_0 [-]"; p301 "ebs_sBSP_stCMaxInValve_Rear_Right (init) export=true name=ebs_sBSP_stCMaxInValve_Rear_Right prio=1 dataSetName=std dataClassType=initIO dataClassName=initIO unit='-' description='ebs_sBSP_stCMaxInValve_Rear_Right': IO_PNE_Generic.ebs_sBSP_stCMaxInValve_Rear_Right_0 [-]"; p302 "ebs_sBSP_stCMaxOutValve_Rear_Left (init) export=true name=ebs_sBSP_stCMaxOutValve_Rear_Left prio=1 dataSetName=std dataClassType=initIO dataClassName=initIO unit='-' description='ebs_sBSP_stCMaxOutValve_Rear_Left': IO_PNE_Generic.ebs_sBSP_stCMaxOutValve_Rear_Left_0 [-]"; p303 "ebs_sBSP_stCMaxOutValve_Rear_Right (init) export=true name=ebs_sBSP_stCMaxOutValve_Rear_Right prio=1 dataSetName=std dataClassType=initIO dataClassName=initIO unit='-' description='ebs_sBSP_stCMaxOutValve_Rear_Right': IO_PNE_Generic.ebs_sBSP_stCMaxOutValve_Rear_Right_0 [-]"; p304 "ebs_sBSP_stRCMaxInValve_Front, ebs_sBSP_stRCMaxInValve_Front(input) export=true name=ebs_sBSP_stRCMaxInValve_Front prio=1 dataSetName=std dataClassType=initIO dataClassName=initIO unit='-' description='ebs_sBSP_stRCMaxInValve_Front(input)': IO_PNE_Generic.ebs_sBSP_stRCMaxInValve_Front_0 [-]"; p305 "ebs_sBSP_stRCMaxInValve_Rear, ebs_sBSP_stRCMaxInValve_Rear(input) export=true name=ebs_sBSP_stRCMaxInValve_Rear prio=1 dataSetName=std dataClassType=initIO dataClassName=initIO unit='-' description='ebs_sBSP_stRCMaxInValve_Rear(input)': IO_PNE_Generic.ebs_sBSP_stRCMaxInValve_Rear_0 [-]"; p306 "ebs_sBSP_stRCMaxOutValve_Front, ebs_sBSP_stRCMaxOutValve_Front(input) export=true name=ebs_sBSP_stRCMaxOutValve_Front prio=1 dataSetName=std dataClassType=initIO dataClassName=initIO unit='-' description='ebs_sBSP_stRCMaxOutValve_Front(input)': IO_PNE_Generic.ebs_sBSP_stRCMaxOutValve_Front_0 [-]"; p307 "ebs_sBSP_stRCMaxOutValve_Rear, ebs_sBSP_stRCMaxOutValve_Rear(input) export=true name=ebs_sBSP_stRCMaxOutValve_Rear prio=1 dataSetName=std dataClassType=initIO dataClassName=initIO unit='-' description='ebs_sBSP_stRCMaxOutValve_Rear(input)': IO_PNE_Generic.ebs_sBSP_stRCMaxOutValve_Rear_0 [-]"; p308 "ebs_sBSP_stTCVBuValve (init) export=true name=ebs_sBSP_stTCVBuValve prio=1 dataSetName=std dataClassType=initIO dataClassName=initIO unit='-' description='ebs_sBSP_stTCVBuValv': IO_PNE_Generic.ebs_sBSP_stTCVBuValve_0 [-]"; p309 "ebs_sBSP_stTCVInValve (init) export=true name=ebs_sBSP_stTCVInValve prio=1 dataSetName=std dataClassType=initIO dataClassName=initIO unit='-' description='ebs_sBSP_stTCVInValve': IO_PNE_Generic.ebs_sBSP_stTCVInValve_0 [-]"; p310 "ebs_sBSP_stTCVOutValve (init) export=true name=ebs_sBSP_stTCVOutValve prio=1 dataSetName=std dataClassType=initIO dataClassName=initIO unit='-' description='ebs_sBSP_stTCVOutValve': IO_PNE_Generic.ebs_sBSP_stTCVOutValve_0 [-]"; p311 "ebs_sil_AAle_force (init) export=true name=ebs_sil_AAle_force prio=1 dataSetName=std dataClassType=initIO dataClassName=initIO unit='N' description='ebs_sil_AAle_force': IO_PNE_Generic.ebs_sil_AAle_force_0 [-]"; p312 "ebs_sil_AAle_vel (init) export=true name=ebs_sil_AAle_vel prio=1 dataSetName=std dataClassType=initIO dataClassName=initIO unit='m/s' description='ebs_sil_AAle_vel': IO_PNE_Generic.ebs_sil_AAle_vel_0 [-]"; p313 "ebs_sil_AAri_force (init) export=true name=ebs_sil_AAri_force prio=1 dataSetName=std dataClassType=initIO dataClassName=initIO unit='N' description='ebs_sil_AAri_force': IO_PNE_Generic.ebs_sil_AAri_force_0 [-]"; p314 "ebs_sil_AAri_vel (init) export=true name=ebs_sil_AAri_vel prio=1 dataSetName=std dataClassType=initIO dataClassName=initIO unit='m/s' description='ebs_sil_AAri_vel': IO_PNE_Generic.ebs_sil_AAri_vel_0 [-]"; p315 "ebs_sil_FAle_force (init) export=true name=ebs_sil_FAle_force prio=1 dataSetName=std dataClassType=initIO dataClassName=initIO unit='N' description='ebs_sil_FAle_force': IO_PNE_Generic.ebs_sil_FAle_force_0 [-]"; p316 "ebs_sil_FAle_vel (init) export=true name=ebs_sil_FAle_vel prio=1 dataSetName=std dataClassType=initIO dataClassName=initIO unit='m/s' description='ebs_sil_FAle_vel': IO_PNE_Generic.ebs_sil_FAle_vel_0 [-]"; p317 "ebs_sil_FAri_force (init) export=true name=ebs_sil_FAri_force prio=1 dataSetName=std dataClassType=initIO dataClassName=initIO unit='N' description='ebs_sil_FAri_force': IO_PNE_Generic.ebs_sil_FAri_force_0 [-]"; p318 "ebs_sil_FAri_vel (init) export=true name=ebs_sil_FAri_vel prio=1 dataSetName=std dataClassType=initIO dataClassName=initIO unit='m/s' description='ebs_sil_FAri_vel': IO_PNE_Generic.ebs_sil_FAri_vel_0 [-]"; p319 "ebs_sil_RAle_force (init) export=true name=ebs_sil_RAle_force prio=1 dataSetName=std dataClassType=initIO dataClassName=initIO unit='N' description='ebs_sil_RAle_force': IO_PNE_Generic.ebs_sil_RAle_force_0 [-]"; p320 "ebs_sil_RAle_vel (init) export=true name=ebs_sil_RAle_vel prio=1 dataSetName=std dataClassType=initIO dataClassName=initIO unit='m/s' description='ebs_sil_RAle_vel': IO_PNE_Generic.ebs_sil_RAle_vel_0 [-]"; p321 "ebs_sil_RAri_force (init) export=true name=ebs_sil_RAri_force prio=1 dataSetName=std dataClassType=initIO dataClassName=initIO unit='N' description='ebs_sil_RAri_force': IO_PNE_Generic.ebs_sil_RAri_force_0 [-]"; p322 "ebs_sil_RAri_vel (init) export=true name=ebs_sil_RAri_vel prio=1 dataSetName=std dataClassType=initIO dataClassName=initIO unit='m/s' description='ebs_sil_RAri_vel': IO_PNE_Generic.ebs_sil_RAri_vel_0 [-]"; p323 "ebs_st3by2_First (init) export=true name=ebs_st3by2_First prio=1 dataSetName=std dataClassType=initIO dataClassName=initIO unit='-' description='ebs_st3by2_First': IO_PNE_Generic.ebs_st3by2_First_0 [-]"; p324 "ebs_st3by2_Second (init) export=true name=ebs_st3by2_Second prio=1 dataSetName=std dataClassType=initIO dataClassName=initIO unit='-' description='ebs_st3by2_Second': IO_PNE_Generic.ebs_st3by2_Second_0 [-]"; p325 "ebs_TCV_pDmd (init) export=true name=ebs_TCV_pDmd prio=1 dataSetName=std dataClassType=initIO dataClassName=initIO unit='-' description='ebs_TCV_pDmd': IO_PNE_Generic.ebs_TCV_pDmd_0 [-]"; p326 "env_air_frontVel export=true name=env_air_frontVel prio=1 dataSetName=std dataClassType=initIO dataClassName=initIO unit=m/s description='env_air_frontVel': IO_PNE_Generic.env_air_frontVel_0 [-]"; p327 "amb air pressure (init) export=true name=env_pressure prio=1 dataSetName=std dataClassType=initIO dataClassName=initIO unit=mbar description='env_pressure': IO_PNE_Generic.env_pressure_0 [-]"; p328 "amb air Temperature (init) export=true name=env_Temperature prio=1 dataSetName=std dataClassType=initIO dataClassName=initIO unit=degC description='env_Temperature': IO_PNE_Generic.env_Temperature_0 [-]"; p329 "Failure_electric_circuit_AA (init) export=true name=Failure_electric_circuit_AA prio=1 dataSetName=std dataClassType=initIO dataClassName=initIO unit='-' description='Failure_electric_circuit_AA': IO_PNE_Generic.Failure_electric_circuit_AA_0 [-]"; p330 "Failure_electric_circuit_FA (init) export=true name=Failure_electric_circuit_FA prio=1 dataSetName=std dataClassType=initIO dataClassName=initIO unit='-' description='Failure_electric_circuit_FA': IO_PNE_Generic.Failure_electric_circuit_FA_0 [-]"; p331 "Failure_electric_circuit_RA (init) export=true name=Failure_electric_circuit_RA prio=1 dataSetName=std dataClassType=initIO dataClassName=initIO unit='-' description='Failure_electric_circuit_RA': IO_PNE_Generic.Failure_electric_circuit_RA_0 [-]"; p332 "Failure_pneumatic_circuit_FA (init) export=true name=Failure_pneumatic_circuit_FA prio=1 dataSetName=std dataClassType=initIO dataClassName=initIO unit='-' description='Failure_pneumatic_circuit_FA': IO_PNE_Generic.Failure_pneumatic_circuit_FA_0 [-]"; p333 "Failure_pneumatic_circuit_RA (init) export=true name=Failure_pneumatic_circuit_RA prio=1 dataSetName=std dataClassType=initIO dataClassName=initIO unit='-' description='Failure_pneumatic_circuit_RA': IO_PNE_Generic.Failure_pneumatic_circuit_RA_0 [-]"; p334 "pne_AirConsumptionFlow_AirSuspension (init) export=true name=pne_AirConsumptionFlow_AirSuspension prio=1 dataSetName=std dataClassType=initIO dataClassName=initIO unit='barl/s' description='pne_AirConsumptionFlow_AirSuspension': IO_PNE_Generic.pne_AirConsumptionFlow_AirSuspension_0 [-]"; p335 "pne_AirConsumptionFlow_auxiliaries (init) export=true name=pne_AirConsumptionFlow_auxiliaries prio=1 dataSetName=std dataClassType=initIO dataClassName=initIO unit='barl/s' description='pne_AirConsumptionFlow_auxiliaries': IO_PNE_Generic.pne_AirConsumptionFlow_auxiliaries_0 [-]"; p336 "pne_AirConsumptionFlow_doors (init) export=true name=pne_AirConsumptionFlow_doors prio=1 dataSetName=std dataClassType=initIO dataClassName=initIO unit='barl/s' description='pne_AirConsumptionFlow_doors': IO_PNE_Generic.pne_AirConsumptionFlow_doors_0 [-]"; p337 "pne_AirConsumptionFlow_EnduranceBrakes (init) export=true name=pne_AirConsumptionFlow_EnduranceBrakes prio=1 dataSetName=std dataClassType=initIO dataClassName=initIO unit='barl/s' description='pne_AirConsumptionFlow_EnduranceBrakes': IO_PNE_Generic.pne_AirConsumptionFlow_EnduranceBrakes_0 [-]"; p338 "pne_AirConsumptionFlow_engine (init) export=true name=pne_AirConsumptionFlow_engine prio=1 dataSetName=std dataClassType=initIO dataClassName=initIO unit='barl/s' description='pne_AirConsumptionFlow_engine': IO_PNE_Generic.pne_AirConsumptionFlow_engine_0 [-]"; p339 "pne_brk_CompressorInlet_mdot (init) export=true name=pne_AirConsumptionFlow_gearbox prio=1 dataSetName=std dataClassType=initIO dataClassName=initIO unit='barl/s' description='pne_AirConsumptionFlow_gearbox': IO_PNE_Generic.pne_AirConsumptionFlow_gearbox_0 [-]"; p340 "pne_AirConsumptionFlow_leakage (init) export=true name=pne_AirConsumptionFlow_leakage prio=1 dataSetName=std dataClassType=initIO dataClassName=initIO unit='barl/s' description='pne_AirConsumptionFlow_leakage': IO_PNE_Generic.pne_AirConsumptionFlow_leakage_0 [-]"; p341 "pne_AirConsumptionFlow_PowerBoost (init) export=true name=pne_AirConsumptionFlow_PowerBoost prio=1 dataSetName=std dataClassType=initIO dataClassName=initIO unit='barl/s' description='pne_AirConsumptionFlow_PowerBoost': IO_PNE_Generic.pne_AirConsumptionFlow_PowerBoost_0 [-]"; p342 "pne_AirConsumptionFlow_SCR (init) export=true name=pne_AirConsumptionFlow_SCR prio=1 dataSetName=std dataClassType=initIO dataClassName=initIO unit='barl/s' description='pne_AirConsumptionFlow_SCR': IO_PNE_Generic.pne_AirConsumptionFlow_SCR_0 [-]"; p343 "pne_brk_Actual_Pressure_AL (init) export=true name=pne_brk_Actual_Pressure_AL prio=1 dataSetName=std dataClassType=initIO dataClassName=initIO unit=bar description='pne_brk_Actual_Pressure_AL (init)': IO_PNE_Generic.pne_brk_Actual_Pressure_AL_0 [-]"; p344 "pne_brk_Actual_Pressure_AR (init) export=true name=pne_brk_Actual_Pressure_AR prio=1 dataSetName=std dataClassType=initIO dataClassName=initIO unit=bar description='pne_brk_Actual_Pressure_AR (init)': IO_PNE_Generic.pne_brk_Actual_Pressure_AR_0 [-]"; p345 "FrontAxle_pAct (init) export=true name=pne_brk_Actual_Pressure_FA prio=1 dataSetName=std dataClassType=initIO dataClassName=initIO unit=bar description='pne_brk_Actual_Pressure_FA (init)': IO_PNE_Generic.pne_brk_Actual_Pressure_FA_0 [-]"; p346 "pne_brk_Actual_Pressure_FOPB (init), pne_brk_Actual_Pressure_FOPB export=true name=pne_brk_Actual_Pressure_FOPB prio=1 dataSetName=std dataClassType=initIO dataClassName=initIO unit='bar' description='pne_brk_Actual_Pressure_FOPB': IO_PNE_Generic.pne_brk_Actual_Pressure_FOPB_0 [-]"; p347 "pne_brk_Actual_Pressure_Front (init), pne_brk_Actual_Pressure_Front(output) rCMAX export=true name=pne_brk_Actual_Pressure_Front prio=1 dataSetName=std dataClassType=initIO dataClassName=initIO unit='bar' description='pne_brk_Actual_Pressure_Front(output) rCMAX': IO_PNE_Generic.pne_brk_Actual_Pressure_Front_0 [-]"; p348 "pne_brk_Actual_Pressure_Rear (init), pne_brk_Actual_Pressure_Rear(output) rCMAX export=true name=pne_brk_Actual_Pressure_Rear prio=1 dataSetName=std dataClassType=initIO dataClassName=initIO unit='bar' description='pne_brk_Actual_Pressure_Rear(output) rCMAX': IO_PNE_Generic.pne_brk_Actual_Pressure_Rear_0 [-]"; p349 "pne_brk_Actual_Pressure_RL (init) export=true name=pne_brk_Actual_Pressure_RL prio=1 dataSetName=std dataClassType=initIO dataClassName=initIO unit=bar description='pne_brk_Actual_Pressure_RL (init)': IO_PNE_Generic.pne_brk_Actual_Pressure_RL_0 [-]"; p350 "pne_brk_Actual_Pressure_RR (init) export=true name=pne_brk_Actual_Pressure_RR prio=1 dataSetName=std dataClassType=initIO dataClassName=initIO unit=bar description='pne_brk_Actual_Pressure_RR (init)': IO_PNE_Generic.pne_brk_Actual_Pressure_RR_0 [-]"; p351 "pne_brk_Actual_Pressure_TCV (init) export=true name=pne_brk_Actual_Pressure_TCV prio=1 dataSetName=std dataClassType=initIO dataClassName=initIO unit=bar description='pne_brk_Actual_Pressure_TCV (init)': IO_PNE_Generic.pne_brk_Actual_Pressure_TCV_0 [-]"; p352 "pne_brk_AdditionalAxle_AxMo_left_rotVel (init) export=true name=pne_brk_AdditionalAxle_AxMo_left_rotVel prio=1 dataSetName=std dataClassType=initIO dataClassName=initIO unit=rad/s description='pne_brk_AdditionalAxle_AxMo_left_rotVel (init)': IO_PNE_Generic.pne_brk_AdditionalAxle_AxMo_left_rotVel_0 [-]"; p353 "pne_brk_AdditionalAxle_AxMo_right_rotVel (init) export=true name=pne_brk_AdditionalAxle_AxMo_right_rotVel prio=1 dataSetName=std dataClassType=initIO dataClassName=initIO unit=rad/s description='pne_brk_AdditionalAxle_AxMo_right_rotVel (init)': IO_PNE_Generic.pne_brk_AdditionalAxle_AxMo_right_rotVel_0 [-]"; p354 "pne_brk_AdditionalAxle_left_pAct (init) export=true name=pne_brk_AdditionalAxle_left_pAct prio=1 dataSetName=std dataClassType=initIO dataClassName=initIO unit=bar description='pne_brk_AdditionalAxle_left_pAct (init)': IO_PNE_Generic.pne_brk_AdditionalAxle_left_pAct_0 [-]"; p355 "pne_brk_AdditionalAxle_left_rotVel (init) export=true name=pne_brk_AdditionalAxle_left_rotVel prio=1 dataSetName=std dataClassType=initIO dataClassName=initIO unit=rad/s description='pne_brk_AdditionalAxle_left_rotVel (init)': IO_PNE_Generic.pne_brk_AdditionalAxle_left_rotVel_0 [-]"; p356 "pne_brk_AdditionalAxle_right_pAct (init) export=true name=pne_brk_AdditionalAxle_right_pAct prio=1 dataSetName=std dataClassType=initIO dataClassName=initIO unit=bar description='pne_brk_AdditionalAxle_right_pAct (init)': IO_PNE_Generic.pne_brk_AdditionalAxle_right_pAct_0 [-]"; p357 "pne_brk_AdditionalAxle_right_rotVel (init) export=true name=pne_brk_AdditionalAxle_right_rotVel prio=1 dataSetName=std dataClassType=initIO dataClassName=initIO unit=rad/s description='pne_brk_AdditionalAxle_right_rotVel (init)': IO_PNE_Generic.pne_brk_AdditionalAxle_right_rotVel_0 [-]"; p358 "Air Compressor - angular acceleration (init) export=true name=pne_brk_AirCompressor_angAcc prio=1 dataSetName=std dataClassType=initIO dataClassName=initIO unit=rad/s^2 description='Air Compressor - angular acceleration (init)': IO_PNE_Generic.pne_brk_AirCompressor_angAcc_0 [-]"; p359 "Air Compressor - angular position (init) export=true name=pne_brk_AirCompressor_angPos prio=1 dataSetName=std dataClassType=initIO dataClassName=initIO unit=rad description='Air Compressor - angular position (init)': IO_PNE_Generic.pne_brk_AirCompressor_angPos_0 [-]"; p360 "Air Compressor - angular velocity with gear ratio iAirCompr 1.412 (init) export=true name=pne_brk_AirCompressor_angVel prio=1 dataSetName=std dataClassType=initIO dataClassName=initIO unit=rad/s description='Air Compressor - angular velocity with gear ratio iAirCompr 1.412 (init)': IO_PNE_Generic.pne_brk_AirCompressor_angVel_0 [-]"; p361 "pne_brk_AirCompressor_delivery (init) export=true name=pne_brk_AirCompressor_delivery prio=1 dataSetName=std dataClassType=initIO dataClassName=initIO unit='l/min' description='pne_brk_AirCompressor_delivery': IO_PNE_Generic.pne_brk_AirCompressor_delivery_0 [-]"; p362 "pne_brk_AirCompressor_torque [Nm] (init) export=true name=pne_brk_AirCompressor_torque prio=1 dataSetName=std dataClassType=initIO dataClassName=initIO unit=Nm description='pne_brk_AirCompressor_torque [Nm] (init)': IO_PNE_Generic.pne_brk_AirCompressor_torque_0 [-]"; p363 "pne_brk_AirConsumpEng_massfracH2O (init) export=true name=pne_brk_AirConsumpEng_massfracH2O prio=1 dataSetName=std dataClassType=initIO dataClassName=initIO unit='-' description='pne_brk_AirConsumpEng_massfracH2O (init)': IO_PNE_Generic.pne_brk_AirConsumpEng_massfracH2O_0 [-]"; p364 "pne_brk_AirConsumpEng_mdot (init) export=true name=pne_brk_AirConsumpEng_mdot prio=1 dataSetName=std dataClassType=initIO dataClassName=initIO unit=kg/s description='pne_brk_AirConsumpEng_mdot': IO_PNE_Generic.pne_brk_AirConsumpEng_mdot_0 [-]"; p365 "pne_brk_AirConsumpEng_pressure [mbar] (init) export=true name=pne_brk_AirConsumpEng_pressure prio=1 dataSetName=std dataClassType=initIO dataClassName=initIO unit=mbar description='pne_brk_AirConsumpEng_pressure [mbar] (init) ': IO_PNE_Generic.pne_brk_AirConsumpEng_pressure_0 [-]"; p366 "pne_brk_AirConsumpEng_Temperature [degC] (init) export=true name=pne_brk_AirConsumpEng_Temperature prio=1 dataSetName=std dataClassType=initIO dataClassName=initIO unit=degC description='pne_brk_AirConsumpEng_Temperature [degC] (init)': IO_PNE_Generic.pne_brk_AirConsumpEng_Temperature_0 [-]"; p367 "pne_brk_AirConsumpRet_massfracH2O (init) export=true name=pne_brk_AirConsumpRet_massfracH2O prio=1 dataSetName=std dataClassType=initIO dataClassName=initIO unit='-' description='pne_brk_AirConsumpRet_massfracH2O (init)': IO_PNE_Generic.pne_brk_AirConsumpRet_massfracH2O_0 [-]"; p368 "pne_brk_AirConsumpRet_mdot (init) export=true name=pne_brk_AirConsumpRet_mdot prio=1 dataSetName=std dataClassType=initIO dataClassName=initIO unit=kg/s description='pne_brk_AirConsumpRet_mdot': IO_PNE_Generic.pne_brk_AirConsumpRet_mdot_0 [-]"; p369 "pne_brk_AirConsumpRet_pressure [mbar] (init) export=true name=pne_brk_AirConsumpRet_pressure prio=1 dataSetName=std dataClassType=initIO dataClassName=initIO unit=mbar description='pne_brk_AirConsumpRet_pressure [mbar] (init)': IO_PNE_Generic.pne_brk_AirConsumpRet_pressure_0 [-]"; p370 "pne_brk_AirConsumpRet_Temperature [degC] (init) export=true name=pne_brk_AirConsumpRet_Temperature prio=1 dataSetName=std dataClassType=initIO dataClassName=initIO unit=degC description='pne_brk_AirConsumpRet_Temperature [degC] (init)': IO_PNE_Generic.pne_brk_AirConsumpRet_Temperature_0 [-]"; p371 "pne_brk_AirConsumpTx_massfracH2O (init) export=true name=pne_brk_AirConsumpTx_massfracH2O prio=1 dataSetName=std dataClassType=initIO dataClassName=initIO unit='-' description='pne_brk_AirConsumpTx_massfracH2O (init)': IO_PNE_Generic.pne_brk_AirConsumpTx_massfracH2O_0 [-]"; p372 "pne_brk_AirConsumpTx_mdot (init) export=true name=pne_brk_AirConsumpTx_mdot prio=1 dataSetName=std dataClassType=initIO dataClassName=initIO unit=kg/s description='pne_brk_AirConsumpTx_mdot': IO_PNE_Generic.pne_brk_AirConsumpTx_mdot_0 [-]"; p373 "pne_brk_AirConsumpTx_pressure [mbar] (init) export=true name=pne_brk_AirConsumpTx_pressure prio=1 dataSetName=std dataClassType=initIO dataClassName=initIO unit=mbar description='pne_brk_AirConsumpTx_pressure [mbar] (init)': IO_PNE_Generic.pne_brk_AirConsumpTx_pressure_0 [-]"; p374 "pne_brk_AirConsumpTx_Temperature [degC] (init) export=true name=pne_brk_AirConsumpTx_Temperature prio=1 dataSetName=std dataClassType=initIO dataClassName=initIO unit=degC description='pne_brk_AirConsumpTx_Temperature [degC] (init)': IO_PNE_Generic.pne_brk_AirConsumpTx_Temperature_0 [-]"; p375 "pne_brk_Axle1_BrakingForce_at8p5bar [N] (init) export=true name=pne_brk_Axle1_BrakingForce_at8p5bar prio=1 dataSetName=std dataClassType=initIO dataClassName=initIO unit=N description='pne_brk_Axle1_BrakingForce_at8p5bar [N] (init)': IO_PNE_Generic.pne_brk_Axle1_BrakingForce_at8p5bar_0 [-]"; p376 "pne_brk_Axle1_BrakingPower [kW] (init) export=true name=pne_brk_Axle1_BrakingPower prio=1 dataSetName=std dataClassType=initIO dataClassName=initIO unit=kW description='pne_brk_Axle1_BrakingPower [kW] (init)': IO_PNE_Generic.pne_brk_Axle1_BrakingPower_0 [-]"; p377 "Axle 1 left - angular acceleration (init) export=true name=pne_brk_Axle1_left_angAcc prio=1 dataSetName=std dataClassType=initIO dataClassName=initIO unit=rad/s^2 description='Axle 1 left - angular acceleration (init)': IO_PNE_Generic.pne_brk_Axle1_left_angAcc_0 [-]"; p378 "Axle 1 left - angular position (init) export=true name=pne_brk_Axle1_left_angPos prio=1 dataSetName=std dataClassType=initIO dataClassName=initIO unit=rad description='Axle 1 left - angular position (init)': IO_PNE_Generic.pne_brk_Axle1_left_angPos_0 [-]"; p379 "Axle 1 left - angular velocity (init) export=true name=pne_brk_Axle1_left_angVel prio=1 dataSetName=std dataClassType=initIO dataClassName=initIO unit=rad/s description='Axle 1 left - angular velocity (init)': IO_PNE_Generic.pne_brk_Axle1_left_angVel_0 [-]"; p380 "brake correction coefficient kvT axle 1 left (init) export=true name=pne_brk_Axle1_left_kvT prio=1 dataSetName=std dataClassType=initIO dataClassName=initIO unit='-' description='brake correction coefficient kvT axle 1 left (init)': IO_PNE_Generic.pne_brk_Axle1_left_kvT_0 [-]"; p381 "brake pad thickness axle 1 left (init) export=true name=pne_brk_Axle1_left_sPad_sum prio=1 dataSetName=std dataClassType=initIO dataClassName=initIO unit=m description='brake pad thickness axle 1 left (init)': IO_PNE_Generic.pne_brk_Axle1_left_sPad_sum_0 [-]"; p382 "axle 1 left temperature of the cooling surface area [degC] (init) export=true name=pne_brk_Axle1_left_Tcooldown prio=1 dataSetName=std dataClassType=initIO dataClassName=initIO unit=degC description='axle 1 left temperature of the cooling surface area [degC] (init)': IO_PNE_Generic.pne_brk_Axle1_left_Tcooldown_0 [-]"; p383 "axle 1 left temperature of the friction area [degC] (init) export=true name=pne_brk_Axle1_left_Tfriction prio=1 dataSetName=std dataClassType=initIO dataClassName=initIO unit=degC description='axle 1 left temperature of the friction area [degC] (init)': IO_PNE_Generic.pne_brk_Axle1_left_Tfriction_0 [-]"; p384 "axle 1 left temperature of the friction area [degC] (init) export=true name=pne_brk_Axle1_left_Tinterior prio=1 dataSetName=std dataClassType=initIO dataClassName=initIO unit=degC description='axle 1 left inner temperature [degC] (init)': IO_PNE_Generic.pne_brk_Axle1_left_Tinterior_0 [-]"; p385 "pne_brk_Axle1_left_torque [Nm] (init) export=true name=pne_brk_Axle1_left_torque prio=1 dataSetName=std dataClassType=initIO dataClassName=initIO unit=Nm description='pne_brk_Axle1_left_torque [Nm] (init)': IO_PNE_Generic.pne_brk_Axle1_left_torque_0 [-]"; p386 "pne_brk_Axle1_left_torque_grinding [Nm] (init) export=true name=pne_brk_Axle1_left_torque_grinding prio=1 dataSetName=std dataClassType=initIO dataClassName=initIO unit=Nm description='pne_brk_Axle1_right_torque [Nm] (init)': IO_PNE_Generic.pne_brk_Axle1_left_torque_grinding_0 [-]"; p387 "Axle 1 right - angular acceleration (init) export=true name=pne_brk_Axle1_right_angAcc prio=1 dataSetName=std dataClassType=initIO dataClassName=initIO unit=rad/s^2 description='Axle 1 right - angular acceleration (init)': IO_PNE_Generic.pne_brk_Axle1_right_angAcc_0 [-]"; p388 "Axle 1 right - angular position (init) export=true name=pne_brk_Axle1_right_angPos prio=1 dataSetName=std dataClassType=initIO dataClassName=initIO unit=rad description='Axle 1 right - angular position (init)': IO_PNE_Generic.pne_brk_Axle1_right_angPos_0 [-]"; p389 "Axle 1 right - angular velocity (init) export=true name=pne_brk_Axle1_right_angVel prio=1 dataSetName=std dataClassType=initIO dataClassName=initIO unit=rad/s description='Axle 1 right - angular velocity (init)': IO_PNE_Generic.pne_brk_Axle1_right_angVel_0 [-]"; p390 "brake correction coefficient kvT axle 1 right (init) export=true name=pne_brk_Axle1_right_kvT prio=1 dataSetName=std dataClassType=initIO dataClassName=initIO unit='-' description='brake correction coefficient kvT axle 1 right (init)': IO_PNE_Generic.pne_brk_Axle1_right_kvT_0 [-]"; p391 "brake pad thickness axle 1 right (init) export=true name=pne_brk_Axle1_right_sPad_sum prio=1 dataSetName=std dataClassType=initIO dataClassName=initIO unit=m description='brake pad thickness axle 1 right (init)': IO_PNE_Generic.pne_brk_Axle1_right_sPad_sum_0 [-]"; p392 "axle 1 right temperature of the cooling surface area [degC] (init) export=true name=pne_brk_Axle1_right_Tcooldown prio=1 dataSetName=std dataClassType=initIO dataClassName=initIO unit=degC description='axle 1 right temperature of the cooling surface area [degC] (init)': IO_PNE_Generic.pne_brk_Axle1_right_Tcooldown_0 [-]"; p393 "axle 1 right temperature of the friction area [degC] (init) export=true name=pne_brk_Axle1_right_Tfriction prio=1 dataSetName=std dataClassType=initIO dataClassName=initIO unit=degC description='axle 1 right temperature of the friction area [degC] (init)': IO_PNE_Generic.pne_brk_Axle1_right_Tfriction_0 [-]"; p394 "axle 1 right temperature of the friction area [degC] (init) export=true name=pne_brk_Axle1_right_Tinterior prio=1 dataSetName=std dataClassType=initIO dataClassName=initIO unit=degC description='axle 1 right inner temperature [degC] (init)': IO_PNE_Generic.pne_brk_Axle1_right_Tinterior_0 [-]"; p395 "pne_brk_Axle1_right_torque [Nm] (init) export=true name=pne_brk_Axle1_right_torque prio=1 dataSetName=std dataClassType=initIO dataClassName=initIO unit=Nm description='pne_brk_Axle1_right_torque [Nm] (init)': IO_PNE_Generic.pne_brk_Axle1_right_torque_0 [-]"; p396 "pne_brk_Axle1_right_torque_grinding [Nm] (init) export=true name=pne_brk_Axle1_right_torque_grinding prio=1 dataSetName=std dataClassType=initIO dataClassName=initIO unit=Nm description='pne_brk_Axle1_right_torque_grinding [Nm] (init)': IO_PNE_Generic.pne_brk_Axle1_right_torque_grinding_0 [-]"; p397 "pne_brk_Axle1_torque_sns [Nm] (init) export=true name=pne_brk_Axle1_torque_sns prio=1 dataSetName=std dataClassType=initIO dataClassName=initIO unit=Nm description='pne_brk_Axle1_torque_sns [Nm] (init)': IO_PNE_Generic.pne_brk_Axle1_torque_sns_0 [-]"; p398 "Cylinder Force Brake Cylinder A1 [N] (init) export=true name=pne_brk_Axle1Brake_Fcyl prio=1 dataSetName=std dataClassType=initIO dataClassName=initIO unit=N description='Cylinder Force Brake Cylinder A1 [N] (init)': IO_PNE_Generic.pne_brk_Axle1Brake_Fcyl_0 [-]"; p399 "Pressure (relative) Brake Cylinder A1 left [bar] (init) export=true name=pne_brk_Axle1Brake_left_pRel prio=1 dataSetName=std dataClassType=initIO dataClassName=initIO unit=bar description='Pressure (relative) Brake Cylinder A1 left [bar] (init)': IO_PNE_Generic.pne_brk_Axle1Brake_left_pRel_0 [-]"; p400 "Pressure (relative) Brake Cylinder A1 right [bar] (init) export=true name=pne_brk_Axle1Brake_right_pRel prio=1 dataSetName=std dataClassType=initIO dataClassName=initIO unit=bar description='Pressure (relative) Brake Cylinder A1 right [bar] (init)': IO_PNE_Generic.pne_brk_Axle1Brake_right_pRel_0 [-]"; p401 "Piston Stroke Brake Cylinder A1 [mm] (init) export=true name=pne_brk_Axle1Brake_stroke prio=1 dataSetName=std dataClassType=initIO dataClassName=initIO unit=mm description='Piston Stroke Brake Cylinder A1 [mm] (init)': IO_PNE_Generic.pne_brk_Axle1Brake_stroke_0 [-]"; p402 "pne_brk_Axle1Brake_Vol [l] (init) export=true name=pne_brk_Axle1Brake_Vol prio=1 dataSetName=std dataClassType=initIO dataClassName=initIO unit=l description='pne_brk_Axle1Brake_Vol [l] (init)': IO_PNE_Generic.pne_brk_Axle1Brake_Vol_0 [-]"; p403 "pne_brk_Axle2_BrakingForce_at8p5bar [N] (init) export=true name=pne_brk_Axle2_BrakingForce_at8p5bar prio=1 dataSetName=std dataClassType=initIO dataClassName=initIO unit=N description='pne_brk_Axle2_BrakingForce_at8p5bar [N] (init)': IO_PNE_Generic.pne_brk_Axle2_BrakingForce_at8p5bar_0 [-]"; p404 "pne_brk_Axle2_BrakingPower [kW] (init) export=true name=pne_brk_Axle2_BrakingPower prio=1 dataSetName=std dataClassType=initIO dataClassName=initIO unit=kW description='pne_brk_Axle2_BrakingPower [kW] (init)': IO_PNE_Generic.pne_brk_Axle2_BrakingPower_0 [-]"; p405 "Axle 2 left - angular acceleration (init) export=true name=pne_brk_Axle2_left_angAcc prio=1 dataSetName=std dataClassType=initIO dataClassName=initIO unit=rad/s^2 description='Axle 2 left - angular acceleration (init)': IO_PNE_Generic.pne_brk_Axle2_left_angAcc_0 [-]"; p406 "Axle 2 left - angular position (init) export=true name=pne_brk_Axle2_left_angPos prio=1 dataSetName=std dataClassType=initIO dataClassName=initIO unit=bar description='Axle 2 left - angular position (init)': IO_PNE_Generic.pne_brk_Axle2_left_angPos_0 [-]"; p407 "Axle 2 left - angular velocity (init) export=true name=pne_brk_Axle2_left_angVel prio=1 dataSetName=std dataClassType=initIO dataClassName=initIO unit=rad/s description='Axle 2 left - angular velocity (init)': IO_PNE_Generic.pne_brk_Axle2_left_angVel_0 [-]"; p408 "brake correction coefficient kvT axle 2 left (init) export=true name=pne_brk_Axle2_left_kvT prio=1 dataSetName=std dataClassType=initIO dataClassName=initIO unit='-' description='brake correction coefficient kvT axle 2 left (init)': IO_PNE_Generic.pne_brk_Axle2_left_kvT_0 [-]"; p409 "brake pad thickness axle 2 left (init) export=true name=pne_brk_Axle2_left_sPad_sum prio=1 dataSetName=std dataClassType=initIO dataClassName=initIO unit=m description='brake pad thickness axle 2 left (init)': IO_PNE_Generic.pne_brk_Axle2_left_sPad_sum_0 [-]"; p410 "axle 2 left temperature of the cooling surface area [degC] (init) export=true name=pne_brk_Axle2_left_Tcooldown prio=1 dataSetName=std dataClassType=initIO dataClassName=initIO unit=degC description='axle 2 left temperature of the cooling surface area [degC] (init)': IO_PNE_Generic.pne_brk_Axle2_left_Tcooldown_0 [-]"; p411 "axle 2 left temperature of the friction area [degC] (init) export=true name=pne_brk_Axle2_left_Tfriction prio=1 dataSetName=std dataClassType=initIO dataClassName=initIO unit=degC description='axle 2 left temperature of the friction area [degC] (init)': IO_PNE_Generic.pne_brk_Axle2_left_Tfriction_0 [-]"; p412 "axle 2 left temperature of the friction area [degC] (init) export=true name=pne_brk_Axle2_left_Tinterior prio=1 dataSetName=std dataClassType=initIO dataClassName=initIO unit=degC description='axle 2 left inner temperature [degC] (init)': IO_PNE_Generic.pne_brk_Axle2_left_Tinterior_0 [-]"; p413 "pne_brk_Axle2_left_torque [Nm] (init) export=true name=pne_brk_Axle2_left_torque prio=1 dataSetName=std dataClassType=initIO dataClassName=initIO unit=Nm description='pne_brk_Axle2_left_torque [Nm] (init)': IO_PNE_Generic.pne_brk_Axle2_left_torque_0 [-]"; p414 "pne_brk_Axle2_left_torque_grinding [Nm] (init) export=true name=pne_brk_Axle2_left_torque_grinding prio=1 dataSetName=std dataClassType=initIO dataClassName=initIO unit=Nm description='pne_brk_Axle2_left_torque_grinding [Nm] (init)': IO_PNE_Generic.pne_brk_Axle2_left_torque_grinding_0 [-]"; p415 "Axle 2 right - angular acceleration (init) export=true name=pne_brk_Axle2_right_angAcc prio=1 dataSetName=std dataClassType=initIO dataClassName=initIO unit=rad/s^2 description='Axle 2 right - angular acceleration (init)': IO_PNE_Generic.pne_brk_Axle2_right_angAcc_0 [-]"; p416 "Axle 2 right - angular position (init) export=true name=pne_brk_Axle2_right_angPos prio=1 dataSetName=std dataClassType=initIO dataClassName=initIO unit=bar description='Axle 2 right - angular position (init)': IO_PNE_Generic.pne_brk_Axle2_right_angPos_0 [-]"; p417 "Axle 2 right - angular velocity (init) export=true name=pne_brk_Axle2_right_angVel prio=1 dataSetName=std dataClassType=initIO dataClassName=initIO unit=rad/s description='Axle 2 right - angular velocity (init)': IO_PNE_Generic.pne_brk_Axle2_right_angVel_0 [-]"; p418 "brake correction coefficient kvT axle 2 right (init) export=true name=pne_brk_Axle2_right_kvT prio=1 dataSetName=std dataClassType=initIO dataClassName=initIO unit='-' description='brake correction coefficient kvT axle 2 right (init)': IO_PNE_Generic.pne_brk_Axle2_right_kvT_0 [-]"; p419 "brake pad thickness axle 2 right (init) export=true name=pne_brk_Axle2_right_sPad_sum prio=1 dataSetName=std dataClassType=initIO dataClassName=initIO unit=m description='brake pad thickness axle 2 right (init)': IO_PNE_Generic.pne_brk_Axle2_right_sPad_sum_0 [-]"; p420 "axle 2 right temperature of the cooling surface area [degC] (init) export=true name=pne_brk_Axle2_right_Tcooldown prio=1 dataSetName=std dataClassType=initIO dataClassName=initIO unit=degC description='axle 2 right temperature of the cooling surface area [degC] (init)': IO_PNE_Generic.pne_brk_Axle2_right_Tcooldown_0 [-]"; p421 "axle 2 right temperature of the friction area [degC] (init) export=true name=pne_brk_Axle2_right_Tfriction prio=1 dataSetName=std dataClassType=initIO dataClassName=initIO unit=degC description='axle 2 right temperature of the friction area [degC] (init)': IO_PNE_Generic.pne_brk_Axle2_right_Tfriction_0 [-]"; p422 "axle 2 right temperature of the friction area [degC] (init) export=true name=pne_brk_Axle2_right_Tinterior prio=1 dataSetName=std dataClassType=initIO dataClassName=initIO unit=degC description='axle 2 right inner temperature [degC] (init)': IO_PNE_Generic.pne_brk_Axle2_right_Tinterior_0 [-]"; p423 "pne_brk_Axle2_right_torque [Nm] (init) export=true name=pne_brk_Axle2_right_torque prio=1 dataSetName=std dataClassType=initIO dataClassName=initIO unit=Nm description='pne_brk_Axle2_right_torque [Nm] (init)': IO_PNE_Generic.pne_brk_Axle2_right_torque_0 [-]"; p424 "pne_brk_Axle2_right_torque_grinding [Nm] (init) export=true name=pne_brk_Axle2_right_torque_grinding prio=1 dataSetName=std dataClassType=initIO dataClassName=initIO unit=Nm description='pne_brk_Axle2_right_torque_grinding [Nm] (init)': IO_PNE_Generic.pne_brk_Axle2_right_torque_grinding_0 [-]"; p425 "pne_brk_Axle2_torque_sns [Nm] (init) export=true name=pne_brk_Axle2_torque_sns prio=1 dataSetName=std dataClassType=initIO dataClassName=initIO unit=Nm description='pne_brk_Axle2_torque_sns [Nm] (init)': IO_PNE_Generic.pne_brk_Axle2_torque_sns_0 [-]"; p426 "Cylinder Force Brake Cylinder Rear [N] (init) export=true name=pne_brk_Axle2Brake_Fcyl prio=1 dataSetName=std dataClassType=initIO dataClassName=initIO unit=N description='Cylinder Force Brake Cylinder Rear [N] (init)': IO_PNE_Generic.pne_brk_Axle2Brake_Fcyl_0 [-]"; p427 "Pressure (relative) Brake Cylinder A2 left [bar] (init) export=true name=pne_brk_Axle2Brake_left_pRel prio=1 dataSetName=std dataClassType=initIO dataClassName=initIO unit=bar description='Pressure (relative) Brake Cylinder A2 left [bar] (init)': IO_PNE_Generic.pne_brk_Axle2Brake_left_pRel_0 [-]"; p428 "Pressure (relative) Brake Cylinder A2 right [bar] (init) export=true name=pne_brk_Axle2Brake_right_pRel prio=1 dataSetName=std dataClassType=initIO dataClassName=initIO unit=bar description='Pressure (relative) Brake Cylinder A2 right [bar] (init)': IO_PNE_Generic.pne_brk_Axle2Brake_right_pRel_0 [-]"; p429 "Piston Stroke Brake Cylinder A2 [mm] (init) export=true name=pne_brk_Axle2Brake_stroke prio=1 dataSetName=std dataClassType=initIO dataClassName=initIO unit=mm description='Piston Stroke Brake Cylinder A2 [mm] (init)': IO_PNE_Generic.pne_brk_Axle2Brake_stroke_0 [-]"; p430 "pne_brk_Axle2Brake_Vol [l] (init) export=true name=pne_brk_Axle2Brake_Vol prio=1 dataSetName=std dataClassType=initIO dataClassName=initIO unit=l description='pne_brk_Axle2Brake_Vol [l] (init)': IO_PNE_Generic.pne_brk_Axle2Brake_Vol_0 [-]"; p431 "pne_brk_Axle3_BrakingForce_at8p5bar [N] (init) export=true name=pne_brk_Axle3_BrakingForce_at8p5bar prio=1 dataSetName=std dataClassType=initIO dataClassName=initIO unit=N description='pne_brk_Axle3_BrakingForce_at8p5bar [N] (init)': IO_PNE_Generic.pne_brk_Axle3_BrakingForce_at8p5bar_0 [-]"; p432 "pne_brk_Axle3_BrakingPower [kW] (init) export=true name=pne_brk_Axle3_BrakingPower prio=1 dataSetName=std dataClassType=initIO dataClassName=initIO unit=kW description='pne_brk_Axle3_BrakingPower [kW] (init)': IO_PNE_Generic.pne_brk_Axle3_BrakingPower_0 [-]"; p433 "Axle 3 left - angular acceleration (init) export=true name=pne_brk_Axle3_left_angAcc prio=1 dataSetName=std dataClassType=initIO dataClassName=initIO unit=rad/s^2 description='Axle 3 left - angular acceleration (init)': IO_PNE_Generic.pne_brk_Axle3_left_angAcc_0 [-]"; p434 "Axle 3 left - angular position (init) export=true name=pne_brk_Axle3_left_angPos prio=1 dataSetName=std dataClassType=initIO dataClassName=initIO unit=bar description='Axle 3 left - angular position (init)': IO_PNE_Generic.pne_brk_Axle3_left_angPos_0 [-]"; p435 "Axle 3 left - angular velocity (init) export=true name=pne_brk_Axle3_left_angVel prio=1 dataSetName=std dataClassType=initIO dataClassName=initIO unit=rad/s description='Axle 3 left - angular velocity (init)': IO_PNE_Generic.pne_brk_Axle3_left_angVel_0 [-]"; p436 "brake correction coefficient kvT axle 3 left (init) export=true name=pne_brk_Axle3_left_kvT prio=1 dataSetName=std dataClassType=initIO dataClassName=initIO unit='-' description='brake correction coefficient kvT axle 3 left (init)': IO_PNE_Generic.pne_brk_Axle3_left_kvT_0 [-]"; p437 "brake pad thickness axle 3 left (init) export=true name=pne_brk_Axle3_left_sPad_sum prio=1 dataSetName=std dataClassType=initIO dataClassName=initIO unit=m description='brake pad thickness axle 3 left (init)': IO_PNE_Generic.pne_brk_Axle3_left_sPad_sum_0 [-]"; p438 "axle 3 left temperature of the cooling surface area [degC] (init) export=true name=pne_brk_Axle3_left_Tcooldown prio=1 dataSetName=std dataClassType=initIO dataClassName=initIO unit=degC description='axle 3 left temperature of the cooling surface area [degC] (init)': IO_PNE_Generic.pne_brk_Axle3_left_Tcooldown_0 [-]"; p439 "axle 3 left temperature of the friction area [degC] (init) export=true name=pne_brk_Axle3_left_Tfriction prio=1 dataSetName=std dataClassType=initIO dataClassName=initIO unit=degC description='axle 3 left temperature of the friction area [degC] (init)': IO_PNE_Generic.pne_brk_Axle3_left_Tfriction_0 [-]"; p440 "axle 3 left temperature of the friction area [degC] (init) export=true name=pne_brk_Axle3_left_Tinterior prio=1 dataSetName=std dataClassType=initIO dataClassName=initIO unit=degC description='axle 3 left inner temperature [degC] (init)': IO_PNE_Generic.pne_brk_Axle3_left_Tinterior_0 [-]"; p441 "pne_brk_Axle3_left_torque [Nm] (init) export=true name=pne_brk_Axle3_left_torque prio=1 dataSetName=std dataClassType=initIO dataClassName=initIO unit=Nm description='pne_brk_Axle3_left_torque [Nm] (init)': IO_PNE_Generic.pne_brk_Axle3_left_torque_0 [-]"; p442 "pne_brk_Axle3_left_torque_grinding [Nm] (init) export=true name=pne_brk_Axle3_left_torque_grinding prio=1 dataSetName=std dataClassType=initIO dataClassName=initIO unit=Nm description='pne_brk_Axle3_left_torque_grinding [Nm] (init)': IO_PNE_Generic.pne_brk_Axle3_left_torque_grinding_0 [-]"; p443 "Axle 3 right - angular acceleration (init) export=true name=pne_brk_Axle3_right_angAcc prio=1 dataSetName=std dataClassType=initIO dataClassName=initIO unit=rad/s^2 description='Axle 3 right - angular acceleration (init)': IO_PNE_Generic.pne_brk_Axle3_right_angAcc_0 [-]"; p444 "Axle 3 right - angular position (init) export=true name=pne_brk_Axle3_right_angPos prio=1 dataSetName=std dataClassType=initIO dataClassName=initIO unit=bar description='Axle 3 right - angular position (init)': IO_PNE_Generic.pne_brk_Axle3_right_angPos_0 [-]"; p445 "Axle 3 right - angular velocity (init) export=true name=pne_brk_Axle3_right_angVel prio=1 dataSetName=std dataClassType=initIO dataClassName=initIO unit=rad/s description='Axle 3 right - angular velocity (init)': IO_PNE_Generic.pne_brk_Axle3_right_angVel_0 [-]"; p446 "brake correction coefficient kvT axle 3 right (init) export=true name=pne_brk_Axle3_right_kvT prio=1 dataSetName=std dataClassType=initIO dataClassName=initIO unit='-' description='brake correction coefficient kvT axle 3 right (init)': IO_PNE_Generic.pne_brk_Axle3_right_kvT_0 [-]"; p447 "brake pad thickness axle 3 right (init) export=true name=pne_brk_Axle3_right_sPad_sum prio=1 dataSetName=std dataClassType=initIO dataClassName=initIO unit=m description='brake pad thickness axle 3 right (init)': IO_PNE_Generic.pne_brk_Axle3_right_sPad_sum_0 [-]"; p448 "axle 3 right temperature of the cooling surface area [degC] (init) export=true name=pne_brk_Axle3_right_Tcooldown prio=1 dataSetName=std dataClassType=initIO dataClassName=initIO unit=degC description='axle 3 right temperature of the cooling surface area [degC] (init)': IO_PNE_Generic.pne_brk_Axle3_right_Tcooldown_0 [-]"; p449 "axle 3 right temperature of the friction area [degC] (init) export=true name=pne_brk_Axle3_right_Tfriction prio=1 dataSetName=std dataClassType=initIO dataClassName=initIO unit=degC description='axle 3 right temperature of the friction area [degC] (init)': IO_PNE_Generic.pne_brk_Axle3_right_Tfriction_0 [-]"; p450 "axle 3 right temperature of the friction area [degC] (init) export=true name=pne_brk_Axle3_right_Tinterior prio=1 dataSetName=std dataClassType=initIO dataClassName=initIO unit=degC description='axle 3 right inner temperature [degC] (init)': IO_PNE_Generic.pne_brk_Axle3_right_Tinterior_0 [-]"; p451 "pne_brk_Axle3_right_torque [Nm] (init) export=true name=pne_brk_Axle3_right_torque prio=1 dataSetName=std dataClassType=initIO dataClassName=initIO unit=Nm description='pne_brk_Axle3_right_torque [Nm] (init)': IO_PNE_Generic.pne_brk_Axle3_right_torque_0 [-]"; p452 "pne_brk_Axle3_right_torque_grinding [Nm] (init) export=true name=pne_brk_Axle3_right_torque_grinding prio=1 dataSetName=std dataClassType=initIO dataClassName=initIO unit=Nm description='pne_brk_Axle3_right_torque_grinding [Nm] (init)': IO_PNE_Generic.pne_brk_Axle3_right_torque_grinding_0 [-]"; p453 "pne_brk_Axle3_torque_sns [Nm] (init) export=true name=pne_brk_Axle3_torque_sns prio=1 dataSetName=std dataClassType=initIO dataClassName=initIO unit=Nm description='pne_brk_Axle3_torque_sns [Nm] (init)': IO_PNE_Generic.pne_brk_Axle3_torque_sns_0 [-]"; p454 "Cylinder Force Brake Cylinder A3 [N] (init) export=true name=pne_brk_Axle3Brake_Fcyl prio=1 dataSetName=std dataClassType=initIO dataClassName=initIO unit=N description='Cylinder Force Brake Cylinder A3 [N] (init)': IO_PNE_Generic.pne_brk_Axle3Brake_Fcyl_0 [-]"; p455 "Pressure (relative) Brake Cylinder A3 left [bar] (init) export=true name=pne_brk_Axle3Brake_left_pRel prio=1 dataSetName=std dataClassType=initIO dataClassName=initIO unit=bar description='Pressure (relative) Brake Cylinder A3 left [bar] (init)': IO_PNE_Generic.pne_brk_Axle3Brake_left_pRel_0 [-]"; p456 "Pressure (relative) Brake Cylinder A3 right [bar] (init) export=true name=pne_brk_Axle3Brake_right_pRel prio=1 dataSetName=std dataClassType=initIO dataClassName=initIO unit=bar description='Pressure (relative) Brake Cylinder A3 right [bar] (init)': IO_PNE_Generic.pne_brk_Axle3Brake_right_pRel_0 [-]"; p457 "Piston Stroke Brake Cylinder A3 [mm] (init) export=true name=pne_brk_Axle3Brake_stroke prio=1 dataSetName=std dataClassType=initIO dataClassName=initIO unit=mm description='Piston Stroke Brake Cylinder A3 [mm] (init)': IO_PNE_Generic.pne_brk_Axle3Brake_stroke_0 [-]"; p458 "pne_brk_Axle3Brake_Vol [dm3] (init) export=true name=pne_brk_Axle3Brake_Vol prio=1 dataSetName=std dataClassType=initIO dataClassName=initIO unit=l description='pne_brk_Axle3Brake_Vol [dm3] (init)': IO_PNE_Generic.pne_brk_Axle3Brake_Vol_0 [-]"; p459 "pne_brk_Axle4_BrakingForce_at8p5bar [N] (init) export=true name=pne_brk_Axle4_BrakingForce_at8p5bar prio=1 dataSetName=std dataClassType=initIO dataClassName=initIO unit=N description='pne_brk_Axle4_BrakingForce_at8p5bar [N] (init)': IO_PNE_Generic.pne_brk_Axle4_BrakingForce_at8p5bar_0 [-]"; p460 "pne_brk_Axle4_BrakingPower [kW] (init) export=true name=pne_brk_Axle4_BrakingPower prio=1 dataSetName=std dataClassType=initIO dataClassName=initIO unit=kW description='pne_brk_Axle4_BrakingPower [kW] (init)': IO_PNE_Generic.pne_brk_Axle4_BrakingPower_0 [-]"; p461 "Axle 4 left - angular acceleration (init) export=true name=pne_brk_Axle4_left_angAcc prio=1 dataSetName=std dataClassType=initIO dataClassName=initIO unit=rad/s^2 description='Axle 4 left - angular acceleration (init)': IO_PNE_Generic.pne_brk_Axle4_left_angAcc_0 [-]"; p462 "Axle 4 left - angular position (init) export=true name=pne_brk_Axle4_left_angPos prio=1 dataSetName=std dataClassType=initIO dataClassName=initIO unit=bar description='Axle 4 left - angular position (init)': IO_PNE_Generic.pne_brk_Axle4_left_angPos_0 [-]"; p463 "Axle 4 left - angular velocity (init) export=true name=pne_brk_Axle4_left_angVel prio=1 dataSetName=std dataClassType=initIO dataClassName=initIO unit=rad/s description='Axle 4 left - angular velocity (init)': IO_PNE_Generic.pne_brk_Axle4_left_angVel_0 [-]"; p464 "brake correction coefficient kvT axle 4 left (init) export=true name=pne_brk_Axle4_left_kvT prio=1 dataSetName=std dataClassType=initIO dataClassName=initIO unit='-' description='brake correction coefficient kvT axle 4 left (init)': IO_PNE_Generic.pne_brk_Axle4_left_kvT_0 [-]"; p465 "brake pad thickness axle 4 left (init) export=true name=pne_brk_Axle4_left_sPad_sum prio=1 dataSetName=std dataClassType=initIO dataClassName=initIO unit=m description='brake pad thickness axle 4 left (init)': IO_PNE_Generic.pne_brk_Axle4_left_sPad_sum_0 [-]"; p466 "axle 4 left temperature of the cooling surface area [degC] (init) export=true name=pne_brk_Axle4_left_Tcooldown prio=1 dataSetName=std dataClassType=initIO dataClassName=initIO unit=degC description='axle 4 left temperature of the cooling surface area [degC] (init)': IO_PNE_Generic.pne_brk_Axle4_left_Tcooldown_0 [-]"; p467 "axle 4 left temperature of the friction area [degC] (init) export=true name=pne_brk_Axle4_left_Tfriction prio=1 dataSetName=std dataClassType=initIO dataClassName=initIO unit=degC description='axle 4 left temperature of the friction area [degC] (init)': IO_PNE_Generic.pne_brk_Axle4_left_Tfriction_0 [-]"; p468 "axle 4 left temperature of the friction area [degC] (init) export=true name=pne_brk_Axle4_left_Tinterior prio=1 dataSetName=std dataClassType=initIO dataClassName=initIO unit=degC description='axle 4 left inner temperature [degC] (init)': IO_PNE_Generic.pne_brk_Axle4_left_Tinterior_0 [-]"; p469 "pne_brk_Axle4_left_torque [Nm] (init) export=true name=pne_brk_Axle4_left_torque prio=1 dataSetName=std dataClassType=initIO dataClassName=initIO unit=Nm description='pne_brk_Axle4_left_torque [Nm] (init)': IO_PNE_Generic.pne_brk_Axle4_left_torque_0 [-]"; p470 "pne_brk_Axle4_left_torque_grinding [Nm] (init) export=true name=pne_brk_Axle4_left_torque_grinding prio=1 dataSetName=std dataClassType=initIO dataClassName=initIO unit=Nm description='pne_brk_Axle4_left_torque_grinding [Nm] (init)': IO_PNE_Generic.pne_brk_Axle4_left_torque_grinding_0 [-]"; p471 "Axle 4 right - angular acceleration (init) export=true name=pne_brk_Axle4_right_angAcc prio=1 dataSetName=std dataClassType=initIO dataClassName=initIO unit=rad/s^2 description='Axle 4 right - angular acceleration (init)': IO_PNE_Generic.pne_brk_Axle4_right_angAcc_0 [-]"; p472 "Axle 4 right - angular position (init) export=true name=pne_brk_Axle4_right_angPos prio=1 dataSetName=std dataClassType=initIO dataClassName=initIO unit=bar description='Axle 4 right - angular position (init)': IO_PNE_Generic.pne_brk_Axle4_right_angPos_0 [-]"; p473 "Axle 4 right - angular velocity (init) export=true name=pne_brk_Axle4_right_angVel prio=1 dataSetName=std dataClassType=initIO dataClassName=initIO unit=rad/s description='Axle 4 right - angular velocity (init)': IO_PNE_Generic.pne_brk_Axle4_right_angVel_0 [-]"; p474 "brake correction coefficient kvT axle 4 right (init) export=true name=pne_brk_Axle4_right_kvT prio=1 dataSetName=std dataClassType=initIO dataClassName=initIO unit='-' description='brake correction coefficient kvT axle 4 right (init)': IO_PNE_Generic.pne_brk_Axle4_right_kvT_0 [-]"; p475 "brake pad thickness axle 4 right (init) export=true name=pne_brk_Axle4_right_sPad_sum prio=1 dataSetName=std dataClassType=initIO dataClassName=initIO unit=m description='brake pad thickness axle 4 right (init)': IO_PNE_Generic.pne_brk_Axle4_right_sPad_sum_0 [-]"; p476 "axle 4 right temperature of the cooling surface area [degC] (init) export=true name=pne_brk_Axle4_right_Tcooldown prio=1 dataSetName=std dataClassType=initIO dataClassName=initIO unit=degC description='axle 4 right temperature of the cooling surface area [degC] (init)': IO_PNE_Generic.pne_brk_Axle4_right_Tcooldown_0 [-]"; p477 "axle 4 right temperature of the friction area [degC] (init) export=true name=pne_brk_Axle4_right_Tfriction prio=1 dataSetName=std dataClassType=initIO dataClassName=initIO unit=degC description='axle 4 right temperature of the friction area [degC] (init)': IO_PNE_Generic.pne_brk_Axle4_right_Tfriction_0 [-]"; p478 "axle 4 right temperature of the friction area [degC] (init) export=true name=pne_brk_Axle4_right_Tinterior prio=1 dataSetName=std dataClassType=initIO dataClassName=initIO unit=degC description='axle 4 right inner temperature [degC] (init)': IO_PNE_Generic.pne_brk_Axle4_right_Tinterior_0 [-]"; p479 "pne_brk_Axle4_right_torque [Nm] (init) export=true name=pne_brk_Axle4_right_torque prio=1 dataSetName=std dataClassType=initIO dataClassName=initIO unit=Nm description='pne_brk_Axle4_right_torque [Nm] (init)': IO_PNE_Generic.pne_brk_Axle4_right_torque_0 [-]"; p480 "pne_brk_Axle4_right_torque_grinding [Nm] (init) export=true name=pne_brk_Axle4_right_torque_grinding prio=1 dataSetName=std dataClassType=initIO dataClassName=initIO unit=Nm description='pne_brk_Axle4_right_torque_grinding [Nm] (init)': IO_PNE_Generic.pne_brk_Axle4_right_torque_grinding_0 [-]"; p481 "pne_brk_Axle4_torque_sns [Nm] (init) export=true name=pne_brk_Axle4_torque_sns prio=1 dataSetName=std dataClassType=initIO dataClassName=initIO unit=Nm description='pne_brk_Axle4_torque_sns [Nm] (init)': IO_PNE_Generic.pne_brk_Axle4_torque_sns_0 [-]"; p482 "Cylinder Force Brake Cylinder A4 [N] (init) export=true name=pne_brk_Axle4Brake_Fcyl prio=1 dataSetName=std dataClassType=initIO dataClassName=initIO unit=N description='Cylinder Force Brake Cylinder A4 [N] (init)': IO_PNE_Generic.pne_brk_Axle4Brake_Fcyl_0 [-]"; p483 "Pressure (relative) Brake Cylinder A4 left [bar] (init) export=true name=pne_brk_Axle4Brake_left_pRel prio=1 dataSetName=std dataClassType=initIO dataClassName=initIO unit=bar description='Pressure (relative) Brake Cylinder A4 left [bar] (init)': IO_PNE_Generic.pne_brk_Axle4Brake_left_pRel_0 [-]"; p484 "Pressure (relative) Brake Cylinder A4 right [bar] (init) export=true name=pne_brk_Axle4Brake_right_pRel prio=1 dataSetName=std dataClassType=initIO dataClassName=initIO unit=bar description='Pressure (relative) Brake Cylinder A4 right [bar] (init)': IO_PNE_Generic.pne_brk_Axle4Brake_right_pRel_0 [-]"; p485 "Piston Stroke Brake Cylinder A4 [mm] (init) export=true name=pne_brk_Axle4Brake_stroke prio=1 dataSetName=std dataClassType=initIO dataClassName=initIO unit=mm description='Piston Stroke Brake Cylinder A4 [mm] (init)': IO_PNE_Generic.pne_brk_Axle4Brake_stroke_0 [-]"; p486 "pne_brk_Axle4Brake_Vol [dm3] (init) export=true name=pne_brk_Axle4Brake_Vol prio=1 dataSetName=std dataClassType=initIO dataClassName=initIO unit=l description='pne_brk_Axle4Brake_Vol [dm3] (init)': IO_PNE_Generic.pne_brk_Axle4Brake_Vol_0 [-]"; p487 "brake pad thickness add. axle left (init) export=true name=pne_brk_BrkWearAALt prio=1 dataSetName=std dataClassType=initIO dataClassName=initIO unit=m description='brake pad thickness trailer axle 3 right (init)': IO_PNE_Generic.pne_brk_BrkWearAALt_0 [-]"; p488 "brake pad thickness add. axle right (init) export=true name=pne_brk_BrkWearAARt prio=1 dataSetName=std dataClassType=initIO dataClassName=initIO unit=m description='brake pad thickness trailer axle 3 right (init)': IO_PNE_Generic.pne_brk_BrkWearAARt_0 [-]"; p489 "brake pad thickness front axle 1 left (init) export=true name=pne_brk_BrkWearFA1Lt prio=1 dataSetName=std dataClassType=initIO dataClassName=initIO unit=m description='brake pad thickness trailer axle 3 right (init)': IO_PNE_Generic.pne_brk_BrkWearFA1Lt_0 [-]"; p490 "brake pad thickness front axle 1 right (init) export=true name=pne_brk_BrkWearFA1Rt prio=1 dataSetName=std dataClassType=initIO dataClassName=initIO unit=m description='brake pad thickness trailer axle 3 right (init)': IO_PNE_Generic.pne_brk_BrkWearFA1Rt_0 [-]"; p491 "brake pad thickness front axle 2 left (init) export=true name=pne_brk_BrkWearFA2Lt prio=1 dataSetName=std dataClassType=initIO dataClassName=initIO unit=m description='brake pad thickness trailer axle 3 right (init)': IO_PNE_Generic.pne_brk_BrkWearFA2Lt_0 [-]"; p492 "brake pad thickness front axle 2 right (init) export=true name=pne_brk_BrkWearFA2Rt prio=1 dataSetName=std dataClassType=initIO dataClassName=initIO unit=m description='brake pad thickness trailer axle 3 right (init)': IO_PNE_Generic.pne_brk_BrkWearFA2Rt_0 [-]"; p493 "brake pad thickness rear axle 1 left (init) export=true name=pne_brk_BrkWearRA1Lt prio=1 dataSetName=std dataClassType=initIO dataClassName=initIO unit=m description='brake pad thickness trailer axle 3 right (init)': IO_PNE_Generic.pne_brk_BrkWearRA1Lt_0 [-]"; p494 "brake pad thickness rear axle 1 right (init) export=true name=pne_brk_BrkWearRA1Rt prio=1 dataSetName=std dataClassType=initIO dataClassName=initIO unit=m description='brake pad thickness trailer axle 3 right (init)': IO_PNE_Generic.pne_brk_BrkWearRA1Rt_0 [-]"; p495 "brake pad thickness rear axle 2 left (init) export=true name=pne_brk_BrkWearRA2Lt prio=1 dataSetName=std dataClassType=initIO dataClassName=initIO unit=m description='brake pad thickness trailer axle 3 right (init)': IO_PNE_Generic.pne_brk_BrkWearRA2Lt_0 [-]"; p496 "brake pad thickness rear axle 2 right (init) export=true name=pne_brk_BrkWearRA2Rt prio=1 dataSetName=std dataClassType=initIO dataClassName=initIO unit=m description='brake pad thickness trailer axle 3 right (init)': IO_PNE_Generic.pne_brk_BrkWearRA2Rt_0 [-]"; p497 "Compressor ON (1 - ON, 0 - OFF) (init) export=true name=pne_brk_CompON prio=1 dataSetName=std dataClassType=initIO dataClassName=initIO unit='-' description='Compressor ON (1 - ON, 0 - OFF) (init)': IO_PNE_Generic.pne_brk_CompON_0 [-]"; p498 "Temperature Compressor Out [degC] (init) export=true name=pne_brk_CompOut_Temp prio=1 dataSetName=std dataClassType=initIO dataClassName=initIO unit=degC description='Temperature Compressor Out [degC] (init)': IO_PNE_Generic.pne_brk_CompOut_Temp_0 [-]"; p499 "massfraction water in gas before compressor (init) export=true name=pne_brk_CompressorInlet_massfracH2O prio=1 dataSetName=std dataClassType=initIO dataClassName=initIO unit='-' description='massfraction water in gas before compressor (init)': IO_PNE_Generic.pne_brk_CompressorInlet_massfracH2O_0 [-]"; p500 "pne_brk_CompressorInlet_mdot (init) export=true name=pne_brk_CompressorInlet_mdot prio=1 dataSetName=std dataClassType=initIO dataClassName=initIO unit=kg/s description='': IO_PNE_Generic.pne_brk_CompressorInlet_mdot_0 [-]"; p501 "pressure before compressor [mbar] (init) export=true name=pne_brk_CompressorInlet_pressure prio=1 dataSetName=std dataClassType=initIO dataClassName=initIO unit=mbar description='pressure before compressor [mbar] (init)': IO_PNE_Generic.pne_brk_CompressorInlet_pressure_0 [-]"; p502 "Temperature before compressor (init) export=true name=pne_brk_CompressorInlet_Temperature prio=1 dataSetName=std dataClassType=initIO dataClassName=initIO unit=degC description='Temperature before compressor (init)': IO_PNE_Generic.pne_brk_CompressorInlet_Temperature_0 [-]"; p503 "Relative Pressure Cooling Pipe [bar] (init) export=true name=pne_brk_CoolingPipe_pRel prio=1 dataSetName=std dataClassType=initIO dataClassName=initIO unit=bar description='Relative Pressure Cooling Pipe [bar] (init)': IO_PNE_Generic.pne_brk_CoolingPipe_pRel_0 [-]"; p504 "Temperature Cooling Pipe [degC] (init) export=true name=pne_brk_CoolingPipe_Temp prio=1 dataSetName=std dataClassType=initIO dataClassName=initIO unit=degC description='Temperature Cooling Pipe [degC] (init)': IO_PNE_Generic.pne_brk_CoolingPipe_Temp_0 [-]"; p505 "Relative Pressure EAPU Input [bar] (init) export=true name=pne_brk_EAPU_pRel prio=1 dataSetName=std dataClassType=initIO dataClassName=initIO unit=bar description='Relative Pressure EAPU Input [bar] (init)': IO_PNE_Generic.pne_brk_EAPU_pRel_0 [-]"; p506 "Temperature EAPU Input [degC] (init) export=true name=pne_brk_EAPU_Temp prio=1 dataSetName=std dataClassType=initIO dataClassName=initIO unit=degC description='Temperature EAPU Input [degC] (init)': IO_PNE_Generic.pne_brk_EAPU_Temp_0 [-]"; p507 "pne_brk_FrontAxle_left_rotVel (init) export=true name=pne_brk_FrontAxle_left_rotVel prio=1 dataSetName=std dataClassType=initIO dataClassName=initIO unit=rad/s description='pne_brk_FrontAxle_left_rotVel(init)': IO_PNE_Generic.pne_brk_FrontAxle_left_rotVel_0 [-]"; p508 "FrontAxle_pAct (init) export=true name=pne_brk_FrontAxle_pAct prio=1 dataSetName=std dataClassType=initIO dataClassName=initIO unit=bar description='FrontAxle_pAct (init)': IO_PNE_Generic.pne_brk_FrontAxle_pAct_0 [-]"; p509 "pne_brk_FrontAxle_right_rotVel (init) export=true name=pne_brk_FrontAxle_right_rotVel prio=1 dataSetName=std dataClassType=initIO dataClassName=initIO unit=rad/s description='pne_brk_FrontAxle_right_rotVel (init)': IO_PNE_Generic.pne_brk_FrontAxle_right_rotVel_0 [-]"; 